simulink model "positionloop1"  (R2024a)
settings: Solver=FixedStepAuto  StartTime=0.0  StopTime=10  FixedStep=1e-4  RelTol=1e-3
values from neighbouring files (symbols this model uses):
  CurrKi = 35.0    [positionloop.sldd]
  CurrKp = 0.17    [positionloop.sldd]
  J = 9.6E-6    [positionloop.sldd]
  Ke = 0.076394372684109757    [positionloop.sldd]
  Kt = 0.132    [positionloop.sldd]
  L = 0.00179    [positionloop.sldd]
  Pn = 8.0    [positionloop.sldd]
  Rs = 1.93    [positionloop.sldd]
  SpdKi = 0.0144    [positionloop.sldd]
  SpdKp = 0.3389    [positionloop.sldd]
  Ts = 0.0001    [positionloop.sldd]
  Udc = 48.0    [positionloop.sldd]
undefined symbols (not defined in the file or in its folder): curr_q_ki, curr_q_kp, I, Jm, K, k_b, k_t, Kd
libraries: slpidlib x33, simulink x8, mcbplantlib x6, autolibpmsmexterior x6, RCTblocks x2
(part 1 of 4)
settings Model: DataDictionary=positionloop.sldd  Creator=Administrator  LastModifiedBy=WuHongrui
settings OptimizationCC: DefaultParameterBehavior=Inlined  UseDivisionForNetSlopeComputation=on  GainParamInheritBuiltInType=on  UseFloatMulNetSlope=on  InlineInvariantSignals=on  PassReuseOutputArgsAs=Individual arguments  ZeroExternalMemoryAtStartup=off  ZeroInternalMemoryAtStartup=off  NoFixptDivByZeroProtection=on  EfficientFloat2IntCast=on  LifeSpan=1  OptimizeBlockOrder=speed  DifferentSizesBufferReuse=on  EfficientTunableParamExpr=on
settings DebuggingCC: ParameterTunabilityLossMsg=error  UnconnectedInputMsg=warning  UnconnectedOutputMsg=warning  UnconnectedLineMsg=warning
settings HardwareCC: ProdBitPerPointer=32  ProdBitPerSizeT=32  ProdBitPerPtrDiffT=32  ProdLargestAtomicInteger=Long  ProdLargestAtomicFloat=Double  ProdWordSize=32  ProdLongLongMode=on  ProdHWDeviceType=ARM Compatible->ARM Cortex-M
settings ModelReferenceCC: EnableRefExpFcnMdlSchedulingChecks=on
settings SFSimCC: MATLABDynamicMemAlloc=off
settings RTWCC: Description=Embedded Coder  SystemTargetFile=ert.tlc  GenCodeOnly=on  PackageGeneratedCodeAndArtifacts=on  TemplateMakefile=ert_default_tmf  GenerateReport=on  LaunchReport=on  GenerateCodeReplacementReport=on  GPUComputeCapability=3.5  DLArmComputeVersion=19.05
settings CodeAppCC: ForceParamTrailComments=on  IgnoreCustomStorageClasses=off  OperatorAnnotations=on  SimulinkDataObjDesc=on  SFDataObjDesc=on  CustomSymbolStrGlobalVar=rt$N$M  CustomSymbolStrType=$N$M  CustomSymbolStrFcn=$N$M$F  CustomSymbolStrMacro=$N$M  InsertBlockDesc=on
settings ERTTargetCC: TargetLangStandard=C99 (ISO)  CodeReplacementLibrary=ARM Cortex-M  GenerateSampleERTMain=on  IncludeMdlTerminateFcn=off  CombineSignalStateStructs=on  SuppressErrorStatus=on  SupportComplex=off  InlinedParameterPlacement=NonHierarchical  ERTCustomFileTemplate=example_file_process.tlc  ERTFilePackagingFormat=CompactWithDataFile

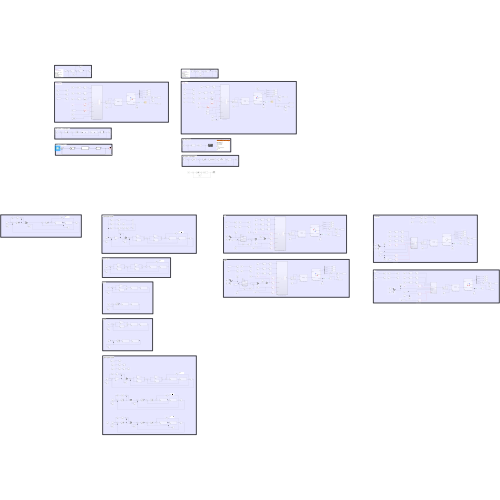
[thumbnail: Simulink's stored preview of the top-level diagram]
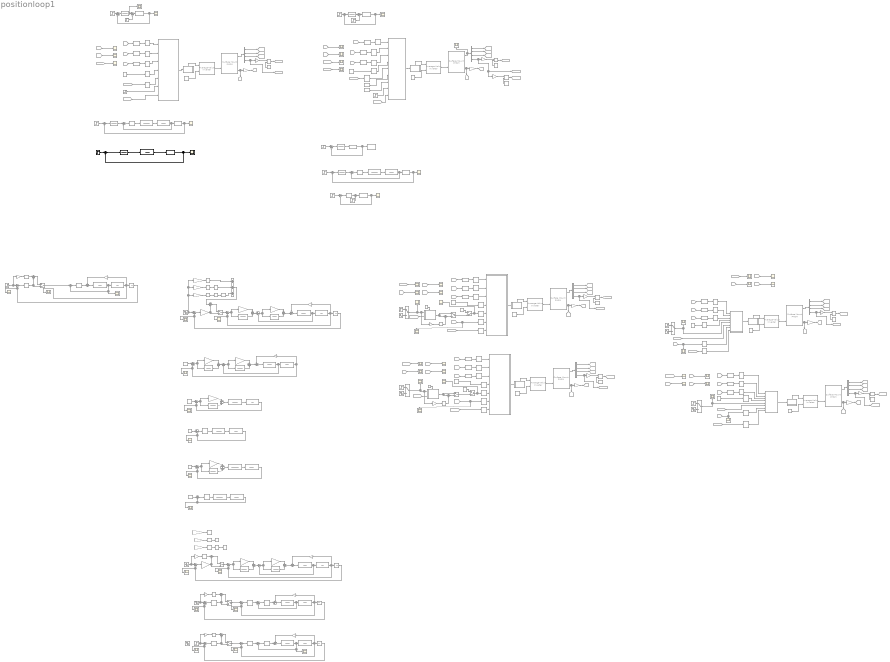
== system positionloop1 ==
  note: 三环
  note: 速度环
  note: S imulate Multiple Random Samples
      | vals = struct();
      | mdl = "positionloop";
      | open_system(mdl);
      | uvars = ufind(mdl);
      | n = 5;
      | for i=1:n
      | vals = usample(uvars);
      | sim(mdl);
      | end
  note: Ke = $\frac{3}{100\pi}Ke^{'}$
  note: Ke = $\frac{3}{100\pi}Ke^{'}$
  note: Ke = $\frac{3}{100\pi}Ke^{'}$
  note: Ke = $\frac{3}{100\pi}Ke^{'}$
  note: 电流环
  note: 速度环+电流环
  note: 位置环+速度环+电流环
  note: 整定
  note: 鲁棒+电流环（考虑减速器？）
  note: 未整定
  note: 系统不确定性仿真
  note: 鲁棒控制
      | （考虑减速器）
      |
      | 执行该仿真前，请打开MATLAB的 mu_synthesis.mlx 文件，运行到第56行，
      | [不确定性参数]之前。
  note: 鲁棒控制
      | （考虑减速器）
  note: 三环+前馈
  note: Ke = $\frac{3}{100\pi}Ke^{'}$
  note: 位置环+速度环+电流环
  note: Ke = $\frac{3}{100\pi}Ke^{'}$
  note: 鲁棒控制
      | （不考虑减速器）
      |
      | 执行该仿真前，请打开MATLAB的 mu_synthesis.mlx 文件，运行到第56行，
      | [不确定性参数]之前。
  note: 鲁棒控制
      | （不考虑减速器）
  note: 鲁棒+电流环（不考虑减速器）
  note: 鲁棒（不考虑减速器）
  Add : Sum  Commented=on  Inputs=+++
  Average-Value Inverter{1..6} (6 alike) : mcbplantlib/Average-Value Inverter  Commented=on
  Bus Selector{1..6} (6 alike) : BusSelector  Commented=on  OutputSignals=IaStator,IbStator,IcStator,MtrPos
  Constant1 : Constant  Commented=on  Value=1.5
  Constant{7,10,12,15,18,21} (6 alike) : Constant  Commented=on  Value=Udc
  Constant{8,11,13,16,19,22} (6 alike) : Constant  Commented=on  Value=Udc  OutDataTypeStr=single
  Constant{5,9,14,17,20,23..24} (7 alike) : Constant  Commented=on  Value=2*pi  OutDataTypeStr=single
  Constant2 : Constant  Commented=on  Value=300
  Constant25 : Constant  Commented=on  Value=0.1  OutDataTypeStr=single
  Constant26 : Constant  Commented=on  Value=0  OutDataTypeStr=single
  Constant3 : Constant  Commented=on
  Constant4 : Constant  Commented=on  Value=300
  Constant6 : Constant  Commented=on  Value=300
  Data Type Conversion{1..9,12..20} (18 alike) : DataTypeConversion  Commented=on  OutDataTypeStr=single  SaturateOnIntegerOverflow=off  RndMeth=Floor
  Derivative{1..18} (18 alike) : Derivative  Commented=on
  From{1,10,13,26,36,48} (6 alike) : From  Commented=on  GotoTag=theta_e  TagVisibility=global
  From{2,9,11,22,30..31,37,40,47,50,57} (11 alike) : From  Commented=on  GotoTag=theta_m  TagVisibility=global
  From{5,12,14,18,23,28,39,43,49,53} (10 alike) : From  Commented=on  GotoTag=W0
  From15 : From  Commented=on  GotoTag=theta_output  TagVisibility=global
  From{3,16,24,32,41,51} (6 alike) : From  Commented=on  GotoTag=ib
  From{4,17,25,33,42,52} (6 alike) : From  Commented=on  GotoTag=ic
  From{6,19,27,34,44,54} (6 alike) : From  Commented=on  GotoTag=Wm
  From{7,20,45,55} (4 alike) : From  Commented=on  GotoTag=theta
  From{8,21,29,35,46,56} (6 alike) : From  Commented=on  GotoTag=ia
  From58 : From  Commented=on  GotoTag=theta_output  TagVisibility=global
  Function-Call Generator1 : simulink/Ports & Subsystems/Function-Call Generator  Commented=on  sample_time=1e-2  numberOfIterations=1  DisallowWideOutput=off
  Function-Call Generator2 : simulink/Ports & Subsystems/Function-Call Generator  Commented=on  sample_time=1e-2  numberOfIterations=1  DisallowWideOutput=off
  Gain{,12..14,17,29} (6 alike) : Gain  Commented=on
  Gain{1,4,10,36} (4 alike) : Gain  Commented=on  Gain=CurrKp
  Gain11 : Gain  Commented=on  Gain=10
  Gain{6..7,15..16,37,39} (6 alike) : Gain  Commented=on  Gain=Ke
  Gain{2,18,20..21,25,27} (6 alike) : Gain  Commented=on  Gain=30/pi  OutDataTypeStr=single
  Gain{3,19,22..23,26,28} (6 alike) : Gain  Commented=on  Gain=Pn  OutDataTypeStr=single
  Gain24 : Gain  Commented=on  Gain=10
  Gain30 : Gain  Commented=on  Gain=L*J/Kt
  Gain31 : Gain  Commented=on  Gain=L*J/Kt
  Gain32 : Gain  Commented=on  Gain=Rs*J/Kt
  Gain33 : Gain  Commented=on  Gain=(Kt+Ke)/Kt
  Gain34 : Gain  Commented=on  Gain=Rs*J/Kt
  Gain35 : Gain  Commented=on  Gain=(Kt+Ke)/Kt
  Gain{5,8..9,38} (4 alike) : Gain  Commented=on  Gain=SpdKp
  Gain40 : Gain  Commented=on  Gain=80  OutDataTypeStr=single
  Goto{,3,12,18,32,39} (6 alike) : Goto  Commented=on  GotoTag=theta_m  TagVisibility=global
  Goto{1,10,15,22,29,36} (6 alike) : Goto  Commented=on  GotoTag=theta_e  TagVisibility=global
  Goto{2,11,17,24,31,38} (6 alike) : Goto  Commented=on  GotoTag=Wm
  Goto{4,13,19,26,33,40} (6 alike) : Goto  Commented=on  GotoTag=W0
  Goto{9,14,16,23,30,37} (6 alike) : Goto  Commented=on  GotoTag=ic
  Goto{5,7,20,27,34,41} (6 alike) : Goto  Commented=on  GotoTag=ia
  Goto{6,8,21,28,35,42} (6 alike) : Goto  Commented=on  GotoTag=ib
  Goto43 : Goto  Commented=on  GotoTag=theta_output  TagVisibility=global
  Integrator{,1..4} (5 alike) : Integrator  Commented=on
  Manual Switch{,1..2,5..8,11..13} (10 alike) : ManualSwitch  Commented=on
  Manual Switch14 : ManualSwitch  Commented=on  CurrentSetting=0
  Manual Switch3 : ManualSwitch  Commented=on  CurrentSetting=0
  Manual Switch4 : ManualSwitch  Commented=on  CurrentSetting=0
  Mod{1..7} (7 alike) : Math  Commented=on  Operator=mod  OutputSignalType=real
  MultiPlot Graph : RCTblocks/MultiPlot Graph  Tag=MultiPlot  Commented=on  tmin=0  tmax=5  ymin=0  ymax=2  vnamesave=multisimout
  PID Controller : slpidlib/PID Controller  Commented=on  Controller=PID  Form=Parallel  TimeDomain=Continuous-time  UseExternalTs=off  SampleTime=-1  IntegratorMethod=Forward Euler  FilterMethod=Forward Euler  ControllerParametersSource=internal  P=0.186  I=0  UseKiTs=off  D=0.087  UseExternalDerivativeSource=off  N=24686.714732734  UseFilter=on  TunerSelectOption=Transfer Function Based (PID Tuner App)  InitialConditionSource=internal  InitialConditionForIntegrator=0  InitialConditionForFilter=0  DifferentiatorICPrevScaledInput=0  ExternalReset=none  TrackingMode=off  Kt=1  LimitOutput=on  SatLimitsSource=internal  UpperSaturationLimit=10  LowerSaturationLimit=-10  LinearizeAsGain=on  AntiWindupMode=none  Kb=1  LimitIntegrator=off  UpperIntegratorSaturationLimit=inf  LowerIntegratorSaturationLimit=-inf  POutMin=[]  POutMax=[]  IOutMin=[]  IOutMax=[]  DOutMin=[]  DOutMax=[]  NOutMin=[]  NOutMax=[]  SumOutMin=[]  SumOutMax=[]  SaturationOutMin=[]  SaturationOutMax=[]  PParamMin=[]  PParamMax=[]  IParamMin=[]  IParamMax=[]  DParamMin=[]  DParamMax=[]  NParamMin=[]  NParamMax=[]  KbParamMin=[]  KbParamMax=[]  KtParamMin=[]  KtParamMax=[]  KbOutMin=[]  KbOutMax=[]  KtOutMin=[]  KtOutMax=[]  IntegratorOutMin=[]  IntegratorOutMax=[]  FilterOutMin=[]  FilterOutMax=[]  SumI1OutMin=[]  SumI1OutMax=[]  SumI2OutMin=[]  SumI2OutMax=[]  SumI3OutMin=[]  SumI3OutMax=[]  SumI4OutMin=[]  SumI4OutMax=[]  SumDOutMin=[]  SumDOutMax=[]  DifferentiatorOutMin=[]  DifferentiatorOutMax=[]  FilterDiffOutCoefMin=[]  FilterDiffOutCoefMax=[]  ReciprocalOutMin=[]  ReciprocalOutMax=[]  SumDenOutMin=[]  SumDenOutMax=[]  SumNumOutMin=[]  SumNumOutMax=[]  DivideOutMin=[]  DivideOutMax=[]  UdiffTsProdOutMin=[]  UdiffTsProdOutMax=[]  NTsProdOutMin=[]  NTsProdOutMax=[]  UintegralTsProdOutMin=[]  UintegralTsProdOutMax=[]  UngainTsProdOutMin=[]  UngainTsProdOutMax=[]  ClampingZeroOutDataTypeStr=Inherit: Inherit via back propagation  ClampingZeroOutMin=[]  ClampingZeroOutMax=[]  FilterDenConstantOutDataTypeStr=Inherit: Inherit via back propagation  FilterDenConstantOutMin=[]  FilterDenConstantOutMax=[]  PCopyOutDataTypeStr=Inherit: Inherit via back propagation  PCopyOutMin=[]  PCopyOutMax=[]  NCopyOutDataTypeStr=Inherit: Inherit via back propagation  NCopyOutMin=[]  NCopyOutMax=[]  IntegratorContinuousStateAttributes=''  IntegratorStateMustResolveToSignalObject=off  IntegratorRTWStateStorageClass=Auto  FilterContinuousStateAttributes=''  FilterStateMustResolveToSignalObject=off  FilterRTWStateStorageClass=Auto  ParallelPVariant=InternalParameters  IdealPVariant=Disabled  IVariant=InternalParameters  DVariant=InternalParameters  IntegratorVariant=Continuous  SatVariant=Enabled  AWVariant=Passthrough  PCopyVariant=Disabled  TRVariant=Disabled  FdbkBlocksVariant=Forward  IdealPFdbkVariant=Disabled  SatFdbkVariant=Disabled  DerivativeFilterVariant=ContFilter  NVariant=InternalParameters  NCopyVariant=Disabled  FilterICVariant=InternalICsFilter  IntegratorICVariant=InternalICs  ExternalResetVariant=Disabled  TRSumVariant=Passthrough  SumFdbkVariant=Disabled  SumVariant=Sum_PID  TsampFilterVariant=InternalTs  TsampNgainVariant=Passthrough  TsampIntegralVariant=Disabled_SignalSpec  ExternalSaturationOutDataTypeStr=Inherit: Same as second input  DerivativeSourceVariant=ErrorSignal
  PID Controller1 : slpidlib/PID Controller  Commented=on  Controller=PI  Form=Parallel  TimeDomain=Continuous-time  UseExternalTs=off  SampleTime=-1  IntegratorMethod=Forward Euler  FilterMethod=Forward Euler  ControllerParametersSource=internal  P=SpdKp  I=SpdKi  UseKiTs=off  D=0  UseExternalDerivativeSource=off  N=100  UseFilter=on  TunerSelectOption=Transfer Function Based (PID Tuner App)  InitialConditionSource=internal  InitialConditionForIntegrator=0  InitialConditionForFilter=0  DifferentiatorICPrevScaledInput=0  ExternalReset=none  TrackingMode=off  Kt=1  LimitOutput=on  SatLimitsSource=internal  UpperSaturationLimit=10  LowerSaturationLimit=-10  LinearizeAsGain=on  AntiWindupMode=none  Kb=1  LimitIntegrator=off  UpperIntegratorSaturationLimit=inf  LowerIntegratorSaturationLimit=-inf  POutMin=[]  POutMax=[]  IOutMin=[]  IOutMax=[]  DOutMin=[]  DOutMax=[]  NOutMin=[]  NOutMax=[]  SumOutMin=[]  SumOutMax=[]  SaturationOutMin=[]  SaturationOutMax=[]  PParamMin=[]  PParamMax=[]  IParamMin=[]  IParamMax=[]  DParamMin=[]  DParamMax=[]  NParamMin=[]  NParamMax=[]  KbParamMin=[]  KbParamMax=[]  KtParamMin=[]  KtParamMax=[]  KbOutMin=[]  KbOutMax=[]  KtOutMin=[]  KtOutMax=[]  IntegratorOutMin=[]  IntegratorOutMax=[]  FilterOutMin=[]  FilterOutMax=[]  SumI1OutMin=[]  SumI1OutMax=[]  SumI2OutMin=[]  SumI2OutMax=[]  SumI3OutMin=[]  SumI3OutMax=[]  SumI4OutMin=[]  SumI4OutMax=[]  SumDOutMin=[]  SumDOutMax=[]  DifferentiatorOutMin=[]  DifferentiatorOutMax=[]  FilterDiffOutCoefMin=[]  FilterDiffOutCoefMax=[]  ReciprocalOutMin=[]  ReciprocalOutMax=[]  SumDenOutMin=[]  SumDenOutMax=[]  SumNumOutMin=[]  SumNumOutMax=[]  DivideOutMin=[]  DivideOutMax=[]  UdiffTsProdOutMin=[]  UdiffTsProdOutMax=[]  NTsProdOutMin=[]  NTsProdOutMax=[]  UintegralTsProdOutMin=[]  UintegralTsProdOutMax=[]  UngainTsProdOutMin=[]  UngainTsProdOutMax=[]  ClampingZeroOutDataTypeStr=Inherit: Inherit via back propagation  ClampingZeroOutMin=[]  ClampingZeroOutMax=[]  FilterDenConstantOutDataTypeStr=Inherit: Inherit via back propagation  FilterDenConstantOutMin=[]  FilterDenConstantOutMax=[]  PCopyOutDataTypeStr=Inherit: Inherit via back propagation  PCopyOutMin=[]  PCopyOutMax=[]  NCopyOutDataTypeStr=Inherit: Inherit via back propagation  NCopyOutMin=[]  NCopyOutMax=[]  IntegratorContinuousStateAttributes=''  IntegratorStateMustResolveToSignalObject=off  IntegratorRTWStateStorageClass=Auto  FilterContinuousStateAttributes=''  FilterStateMustResolveToSignalObject=off  FilterRTWStateStorageClass=Auto  ParallelPVariant=InternalParameters  IdealPVariant=Disabled  IVariant=InternalParameters  DVariant=Disabled  IntegratorVariant=Continuous  SatVariant=Enabled  AWVariant=Passthrough  PCopyVariant=Disabled  TRVariant=Disabled  FdbkBlocksVariant=Forward  IdealPFdbkVariant=Disabled  SatFdbkVariant=Disabled  DerivativeFilterVariant=Disabled  NVariant=Disabled  NCopyVariant=Disabled_SignalSpec  FilterICVariant=Disabled  IntegratorICVariant=InternalICs  ExternalResetVariant=Disabled  TRSumVariant=Passthrough  SumFdbkVariant=Disabled  SumVariant=Sum_PI  TsampFilterVariant=InternalTs  TsampNgainVariant=Passthrough  TsampIntegralVariant=Disabled_SignalSpec  ExternalSaturationOutDataTypeStr=Inherit: Same as second input  DerivativeSourceVariant=Disabled
  PID Controller10 : slpidlib/PID Controller  Commented=on  Controller=P  Form=Parallel  TimeDomain=Continuous-time  UseExternalTs=off  SampleTime=-1  IntegratorMethod=Forward Euler  FilterMethod=Forward Euler  ControllerParametersSource=internal  P=14.0449429845648  I=1.40448915956441e-06  UseKiTs=off  D=0  UseExternalDerivativeSource=off  N=100  UseFilter=on  TunerSelectOption=Transfer Function Based (PID Tuner App)  InitialConditionSource=internal  InitialConditionForIntegrator=0  InitialConditionForFilter=0  DifferentiatorICPrevScaledInput=0  ExternalReset=none  TrackingMode=off  Kt=1  LimitOutput=on  SatLimitsSource=internal  UpperSaturationLimit=Udc*0.9/sqrt(3)  LowerSaturationLimit=-Udc*0.9/sqrt(3)  LinearizeAsGain=on  AntiWindupMode=none  Kb=1  LimitIntegrator=off  UpperIntegratorSaturationLimit=inf  LowerIntegratorSaturationLimit=-inf  POutMin=[]  POutMax=[]  IOutMin=[]  IOutMax=[]  DOutMin=[]  DOutMax=[]  NOutMin=[]  NOutMax=[]  SumOutMin=[]  SumOutMax=[]  SaturationOutMin=[]  SaturationOutMax=[]  PParamMin=[]  PParamMax=[]  IParamMin=[]  IParamMax=[]  DParamMin=[]  DParamMax=[]  NParamMin=[]  NParamMax=[]  KbParamMin=[]  KbParamMax=[]  KtParamMin=[]  KtParamMax=[]  KbOutMin=[]  KbOutMax=[]  KtOutMin=[]  KtOutMax=[]  IntegratorOutMin=[]  IntegratorOutMax=[]  FilterOutMin=[]  FilterOutMax=[]  SumI1OutMin=[]  SumI1OutMax=[]  SumI2OutMin=[]  SumI2OutMax=[]  SumI3OutMin=[]  SumI3OutMax=[]  SumI4OutMin=[]  SumI4OutMax=[]  SumDOutMin=[]  SumDOutMax=[]  DifferentiatorOutMin=[]  DifferentiatorOutMax=[]  FilterDiffOutCoefMin=[]  FilterDiffOutCoefMax=[]  ReciprocalOutMin=[]  ReciprocalOutMax=[]  SumDenOutMin=[]  SumDenOutMax=[]  SumNumOutMin=[]  SumNumOutMax=[]  DivideOutMin=[]  DivideOutMax=[]  UdiffTsProdOutMin=[]  UdiffTsProdOutMax=[]  NTsProdOutMin=[]  NTsProdOutMax=[]  UintegralTsProdOutMin=[]  UintegralTsProdOutMax=[]  UngainTsProdOutMin=[]  UngainTsProdOutMax=[]  ClampingZeroOutDataTypeStr=Inherit: Inherit via back propagation  ClampingZeroOutMin=[]  ClampingZeroOutMax=[]  FilterDenConstantOutDataTypeStr=Inherit: Inherit via back propagation  FilterDenConstantOutMin=[]  FilterDenConstantOutMax=[]  PCopyOutDataTypeStr=Inherit: Inherit via back propagation  PCopyOutMin=[]  PCopyOutMax=[]  NCopyOutDataTypeStr=Inherit: Inherit via back propagation  NCopyOutMin=[]  NCopyOutMax=[]  IntegratorContinuousStateAttributes=''  IntegratorStateMustResolveToSignalObject=off  IntegratorRTWStateStorageClass=Auto  FilterContinuousStateAttributes=''  FilterStateMustResolveToSignalObject=off  FilterRTWStateStorageClass=Auto  ParallelPVariant=InternalParameters  IdealPVariant=Disabled  IVariant=Disabled  DVariant=Disabled  IntegratorVariant=Disabled  SatVariant=Enabled  AWVariant=Disabled  PCopyVariant=Disabled  TRVariant=Disabled  FdbkBlocksVariant=Forward  IdealPFdbkVariant=Disabled  SatFdbkVariant=Disabled  DerivativeFilterVariant=Disabled  NVariant=Disabled  NCopyVariant=Disabled_SignalSpec  FilterICVariant=Disabled  IntegratorICVariant=Disabled  ExternalResetVariant=Disabled  TRSumVariant=Passthrough  SumFdbkVariant=Disabled  SumVariant=Passthrough_P  TsampFilterVariant=InternalTs  TsampNgainVariant=Passthrough  TsampIntegralVariant=Disabled_SignalSpec  ExternalSaturationOutDataTypeStr=Inherit: Same as second input  DerivativeSourceVariant=Disabled
  PID Controller12 : slpidlib/PID Controller  Commented=on  Controller=PI  Form=Parallel  TimeDomain=Continuous-time  UseExternalTs=off  SampleTime=-1  IntegratorMethod=Forward Euler  FilterMethod=Forward Euler  ControllerParametersSource=internal  P=0.0444061130539005  I=8.20535972466433e-05  UseKiTs=off  D=0  UseExternalDerivativeSource=off  N=100  UseFilter=on  TunerSelectOption=Transfer Function Based (PID Tuner App)  InitialConditionSource=internal  InitialConditionForIntegrator=0  InitialConditionForFilter=0  DifferentiatorICPrevScaledInput=0  ExternalReset=none  TrackingMode=off  Kt=1  LimitOutput=on  SatLimitsSource=internal  UpperSaturationLimit=Udc*0.9/sqrt(3)  LowerSaturationLimit=-Udc*0.9/sqrt(3)  LinearizeAsGain=on  AntiWindupMode=none  Kb=1  LimitIntegrator=off  UpperIntegratorSaturationLimit=inf  LowerIntegratorSaturationLimit=-inf  POutMin=[]  POutMax=[]  IOutMin=[]  IOutMax=[]  DOutMin=[]  DOutMax=[]  NOutMin=[]  NOutMax=[]  SumOutMin=[]  SumOutMax=[]  SaturationOutMin=[]  SaturationOutMax=[]  PParamMin=[]  PParamMax=[]  IParamMin=[]  IParamMax=[]  DParamMin=[]  DParamMax=[]  NParamMin=[]  NParamMax=[]  KbParamMin=[]  KbParamMax=[]  KtParamMin=[]  KtParamMax=[]  KbOutMin=[]  KbOutMax=[]  KtOutMin=[]  KtOutMax=[]  IntegratorOutMin=[]  IntegratorOutMax=[]  FilterOutMin=[]  FilterOutMax=[]  SumI1OutMin=[]  SumI1OutMax=[]  SumI2OutMin=[]  SumI2OutMax=[]  SumI3OutMin=[]  SumI3OutMax=[]  SumI4OutMin=[]  SumI4OutMax=[]  SumDOutMin=[]  SumDOutMax=[]  DifferentiatorOutMin=[]  DifferentiatorOutMax=[]  FilterDiffOutCoefMin=[]  FilterDiffOutCoefMax=[]  ReciprocalOutMin=[]  ReciprocalOutMax=[]  SumDenOutMin=[]  SumDenOutMax=[]  SumNumOutMin=[]  SumNumOutMax=[]  DivideOutMin=[]  DivideOutMax=[]  UdiffTsProdOutMin=[]  UdiffTsProdOutMax=[]  NTsProdOutMin=[]  NTsProdOutMax=[]  UintegralTsProdOutMin=[]  UintegralTsProdOutMax=[]  UngainTsProdOutMin=[]  UngainTsProdOutMax=[]  ClampingZeroOutDataTypeStr=Inherit: Inherit via back propagation  ClampingZeroOutMin=[]  ClampingZeroOutMax=[]  FilterDenConstantOutDataTypeStr=Inherit: Inherit via back propagation  FilterDenConstantOutMin=[]  FilterDenConstantOutMax=[]  PCopyOutDataTypeStr=Inherit: Inherit via back propagation  PCopyOutMin=[]  PCopyOutMax=[]  NCopyOutDataTypeStr=Inherit: Inherit via back propagation  NCopyOutMin=[]  NCopyOutMax=[]  IntegratorContinuousStateAttributes=''  IntegratorStateMustResolveToSignalObject=off  IntegratorRTWStateStorageClass=Auto  FilterContinuousStateAttributes=''  FilterStateMustResolveToSignalObject=off  FilterRTWStateStorageClass=Auto  ParallelPVariant=InternalParameters  IdealPVariant=Disabled  IVariant=InternalParameters  DVariant=Disabled  IntegratorVariant=Continuous  SatVariant=Enabled  AWVariant=Passthrough  PCopyVariant=Disabled  TRVariant=Disabled  FdbkBlocksVariant=Forward  IdealPFdbkVariant=Disabled  SatFdbkVariant=Disabled  DerivativeFilterVariant=Disabled  NVariant=Disabled  NCopyVariant=Disabled_SignalSpec  FilterICVariant=Disabled  IntegratorICVariant=InternalICs  ExternalResetVariant=Disabled  TRSumVariant=Passthrough  SumFdbkVariant=Disabled  SumVariant=Sum_PI  TsampFilterVariant=InternalTs  TsampNgainVariant=Passthrough  TsampIntegralVariant=Disabled_SignalSpec  ExternalSaturationOutDataTypeStr=Inherit: Same as second input  DerivativeSourceVariant=Disabled
  PID Controller13 : slpidlib/PID Controller  Commented=on  Controller=PI  Form=Parallel  TimeDomain=Continuous-time  UseExternalTs=off  SampleTime=-1  IntegratorMethod=Forward Euler  FilterMethod=Forward Euler  ControllerParametersSource=internal  P=3.78093167506926  I=4.06645918177242e-07  UseKiTs=off  D=0  UseExternalDerivativeSource=off  N=100  UseFilter=on  TunerSelectOption=Transfer Function Based (PID Tuner App)  InitialConditionSource=internal  InitialConditionForIntegrator=0  InitialConditionForFilter=0  DifferentiatorICPrevScaledInput=0  ExternalReset=none  TrackingMode=off  Kt=1  LimitOutput=on  SatLimitsSource=internal  UpperSaturationLimit=10  LowerSaturationLimit=-10  LinearizeAsGain=on  AntiWindupMode=none  Kb=1  LimitIntegrator=off  UpperIntegratorSaturationLimit=inf  LowerIntegratorSaturationLimit=-inf  POutMin=[]  POutMax=[]  IOutMin=[]  IOutMax=[]  DOutMin=[]  DOutMax=[]  NOutMin=[]  NOutMax=[]  SumOutMin=[]  SumOutMax=[]  SaturationOutMin=[]  SaturationOutMax=[]  PParamMin=[]  PParamMax=[]  IParamMin=[]  IParamMax=[]  DParamMin=[]  DParamMax=[]  NParamMin=[]  NParamMax=[]  KbParamMin=[]  KbParamMax=[]  KtParamMin=[]  KtParamMax=[]  KbOutMin=[]  KbOutMax=[]  KtOutMin=[]  KtOutMax=[]  IntegratorOutMin=[]  IntegratorOutMax=[]  FilterOutMin=[]  FilterOutMax=[]  SumI1OutMin=[]  SumI1OutMax=[]  SumI2OutMin=[]  SumI2OutMax=[]  SumI3OutMin=[]  SumI3OutMax=[]  SumI4OutMin=[]  SumI4OutMax=[]  SumDOutMin=[]  SumDOutMax=[]  DifferentiatorOutMin=[]  DifferentiatorOutMax=[]  FilterDiffOutCoefMin=[]  FilterDiffOutCoefMax=[]  ReciprocalOutMin=[]  ReciprocalOutMax=[]  SumDenOutMin=[]  SumDenOutMax=[]  SumNumOutMin=[]  SumNumOutMax=[]  DivideOutMin=[]  DivideOutMax=[]  UdiffTsProdOutMin=[]  UdiffTsProdOutMax=[]  NTsProdOutMin=[]  NTsProdOutMax=[]  UintegralTsProdOutMin=[]  UintegralTsProdOutMax=[]  UngainTsProdOutMin=[]  UngainTsProdOutMax=[]  ClampingZeroOutDataTypeStr=Inherit: Inherit via back propagation  ClampingZeroOutMin=[]  ClampingZeroOutMax=[]  FilterDenConstantOutDataTypeStr=Inherit: Inherit via back propagation  FilterDenConstantOutMin=[]  FilterDenConstantOutMax=[]  PCopyOutDataTypeStr=Inherit: Inherit via back propagation  PCopyOutMin=[]  PCopyOutMax=[]  NCopyOutDataTypeStr=Inherit: Inherit via back propagation  NCopyOutMin=[]  NCopyOutMax=[]  IntegratorContinuousStateAttributes=''  IntegratorStateMustResolveToSignalObject=off  IntegratorRTWStateStorageClass=Auto  FilterContinuousStateAttributes=''  FilterStateMustResolveToSignalObject=off  FilterRTWStateStorageClass=Auto  ParallelPVariant=InternalParameters  IdealPVariant=Disabled  IVariant=InternalParameters  DVariant=Disabled  IntegratorVariant=Continuous  SatVariant=Enabled  AWVariant=Passthrough  PCopyVariant=Disabled  TRVariant=Disabled  FdbkBlocksVariant=Forward  IdealPFdbkVariant=Disabled  SatFdbkVariant=Disabled  DerivativeFilterVariant=Disabled  NVariant=Disabled  NCopyVariant=Disabled_SignalSpec  FilterICVariant=Disabled  IntegratorICVariant=InternalICs  ExternalResetVariant=Disabled  TRSumVariant=Passthrough  SumFdbkVariant=Disabled  SumVariant=Sum_PI  TsampFilterVariant=InternalTs  TsampNgainVariant=Passthrough  TsampIntegralVariant=Disabled_SignalSpec  ExternalSaturationOutDataTypeStr=Inherit: Same as second input  DerivativeSourceVariant=Disabled
  PID Controller2 : slpidlib/PID Controller  Commented=on  Controller=PI  Form=Parallel  TimeDomain=Continuous-time  UseExternalTs=off  SampleTime=-1  IntegratorMethod=Forward Euler  FilterMethod=Forward Euler  ControllerParametersSource=internal  P=CurrKp  I=CurrKi  UseKiTs=off  D=0  UseExternalDerivativeSource=off  N=100  UseFilter=on  TunerSelectOption=Transfer Function Based (PID Tuner App)  InitialConditionSource=internal  InitialConditionForIntegrator=0  InitialConditionForFilter=0  DifferentiatorICPrevScaledInput=0  ExternalReset=none  TrackingMode=off  Kt=1  LimitOutput=on  SatLimitsSource=internal  UpperSaturationLimit=Udc*0.9/sqrt(3)  LowerSaturationLimit=-Udc*0.9/sqrt(3)  LinearizeAsGain=on  AntiWindupMode=none  Kb=1  LimitIntegrator=off  UpperIntegratorSaturationLimit=inf  LowerIntegratorSaturationLimit=-inf  POutMin=[]  POutMax=[]  IOutMin=[]  IOutMax=[]  DOutMin=[]  DOutMax=[]  NOutMin=[]  NOutMax=[]  SumOutMin=[]  SumOutMax=[]  SaturationOutMin=[]  SaturationOutMax=[]  PParamMin=[]  PParamMax=[]  IParamMin=[]  IParamMax=[]  DParamMin=[]  DParamMax=[]  NParamMin=[]  NParamMax=[]  KbParamMin=[]  KbParamMax=[]  KtParamMin=[]  KtParamMax=[]  KbOutMin=[]  KbOutMax=[]  KtOutMin=[]  KtOutMax=[]  IntegratorOutMin=[]  IntegratorOutMax=[]  FilterOutMin=[]  FilterOutMax=[]  SumI1OutMin=[]  SumI1OutMax=[]  SumI2OutMin=[]  SumI2OutMax=[]  SumI3OutMin=[]  SumI3OutMax=[]  SumI4OutMin=[]  SumI4OutMax=[]  SumDOutMin=[]  SumDOutMax=[]  DifferentiatorOutMin=[]  DifferentiatorOutMax=[]  FilterDiffOutCoefMin=[]  FilterDiffOutCoefMax=[]  ReciprocalOutMin=[]  ReciprocalOutMax=[]  SumDenOutMin=[]  SumDenOutMax=[]  SumNumOutMin=[]  SumNumOutMax=[]  DivideOutMin=[]  DivideOutMax=[]  UdiffTsProdOutMin=[]  UdiffTsProdOutMax=[]  NTsProdOutMin=[]  NTsProdOutMax=[]  UintegralTsProdOutMin=[]  UintegralTsProdOutMax=[]  UngainTsProdOutMin=[]  UngainTsProdOutMax=[]  ClampingZeroOutDataTypeStr=Inherit: Inherit via back propagation  ClampingZeroOutMin=[]  ClampingZeroOutMax=[]  FilterDenConstantOutDataTypeStr=Inherit: Inherit via back propagation  FilterDenConstantOutMin=[]  FilterDenConstantOutMax=[]  PCopyOutDataTypeStr=Inherit: Inherit via back propagation  PCopyOutMin=[]  PCopyOutMax=[]  NCopyOutDataTypeStr=Inherit: Inherit via back propagation  NCopyOutMin=[]  NCopyOutMax=[]  IntegratorContinuousStateAttributes=''  IntegratorStateMustResolveToSignalObject=off  IntegratorRTWStateStorageClass=Auto  FilterContinuousStateAttributes=''  FilterStateMustResolveToSignalObject=off  FilterRTWStateStorageClass=Auto  ParallelPVariant=InternalParameters  IdealPVariant=Disabled  IVariant=InternalParameters  DVariant=Disabled  IntegratorVariant=Continuous  SatVariant=Enabled  AWVariant=Passthrough  PCopyVariant=Disabled  TRVariant=Disabled  FdbkBlocksVariant=Forward  IdealPFdbkVariant=Disabled  SatFdbkVariant=Disabled  DerivativeFilterVariant=Disabled  NVariant=Disabled  NCopyVariant=Disabled_SignalSpec  FilterICVariant=Disabled  IntegratorICVariant=InternalICs  ExternalResetVariant=Disabled  TRSumVariant=Passthrough  SumFdbkVariant=Disabled  SumVariant=Sum_PI  TsampFilterVariant=InternalTs  TsampNgainVariant=Passthrough  TsampIntegralVariant=Disabled_SignalSpec  ExternalSaturationOutDataTypeStr=Inherit: Same as second input  DerivativeSourceVariant=Disabled
  PID Controller3 : slpidlib/PID Controller  Commented=on  Controller=P  Form=Parallel  TimeDomain=Continuous-time  UseExternalTs=off  SampleTime=-1  IntegratorMethod=Forward Euler  FilterMethod=Forward Euler  ControllerParametersSource=internal  P=10  I=SpdKi  UseKiTs=off  D=0  UseExternalDerivativeSource=off  N=100  UseFilter=on  TunerSelectOption=Transfer Function Based (PID Tuner App)  InitialConditionSource=internal  InitialConditionForIntegrator=0  InitialConditionForFilter=0  DifferentiatorICPrevScaledInput=0  ExternalReset=none  TrackingMode=off  Kt=1  LimitOutput=on  SatLimitsSource=internal  UpperSaturationLimit=400  LowerSaturationLimit=-400  LinearizeAsGain=on  AntiWindupMode=none  Kb=1  LimitIntegrator=off  UpperIntegratorSaturationLimit=inf  LowerIntegratorSaturationLimit=-inf  POutMin=[]  POutMax=[]  IOutMin=[]  IOutMax=[]  DOutMin=[]  DOutMax=[]  NOutMin=[]  NOutMax=[]  SumOutMin=[]  SumOutMax=[]  SaturationOutMin=[]  SaturationOutMax=[]  PParamMin=[]  PParamMax=[]  IParamMin=[]  IParamMax=[]  DParamMin=[]  DParamMax=[]  NParamMin=[]  NParamMax=[]  KbParamMin=[]  KbParamMax=[]  KtParamMin=[]  KtParamMax=[]  KbOutMin=[]  KbOutMax=[]  KtOutMin=[]  KtOutMax=[]  IntegratorOutMin=[]  IntegratorOutMax=[]  FilterOutMin=[]  FilterOutMax=[]  SumI1OutMin=[]  SumI1OutMax=[]  SumI2OutMin=[]  SumI2OutMax=[]  SumI3OutMin=[]  SumI3OutMax=[]  SumI4OutMin=[]  SumI4OutMax=[]  SumDOutMin=[]  SumDOutMax=[]  DifferentiatorOutMin=[]  DifferentiatorOutMax=[]  FilterDiffOutCoefMin=[]  FilterDiffOutCoefMax=[]  ReciprocalOutMin=[]  ReciprocalOutMax=[]  SumDenOutMin=[]  SumDenOutMax=[]  SumNumOutMin=[]  SumNumOutMax=[]  DivideOutMin=[]  DivideOutMax=[]  UdiffTsProdOutMin=[]  UdiffTsProdOutMax=[]  NTsProdOutMin=[]  NTsProdOutMax=[]  UintegralTsProdOutMin=[]  UintegralTsProdOutMax=[]  UngainTsProdOutMin=[]  UngainTsProdOutMax=[]  ClampingZeroOutDataTypeStr=Inherit: Inherit via back propagation  ClampingZeroOutMin=[]  ClampingZeroOutMax=[]  FilterDenConstantOutDataTypeStr=Inherit: Inherit via back propagation  FilterDenConstantOutMin=[]  FilterDenConstantOutMax=[]  PCopyOutDataTypeStr=Inherit: Inherit via back propagation  PCopyOutMin=[]  PCopyOutMax=[]  NCopyOutDataTypeStr=Inherit: Inherit via back propagation  NCopyOutMin=[]  NCopyOutMax=[]  IntegratorContinuousStateAttributes=''  IntegratorStateMustResolveToSignalObject=off  IntegratorRTWStateStorageClass=Auto  FilterContinuousStateAttributes=''  FilterStateMustResolveToSignalObject=off  FilterRTWStateStorageClass=Auto  ParallelPVariant=InternalParameters  IdealPVariant=Disabled  IVariant=Disabled  DVariant=Disabled  IntegratorVariant=Disabled  SatVariant=Enabled  AWVariant=Disabled  PCopyVariant=Disabled  TRVariant=Disabled  FdbkBlocksVariant=Forward  IdealPFdbkVariant=Disabled  SatFdbkVariant=Disabled  DerivativeFilterVariant=Disabled  NVariant=Disabled  NCopyVariant=Disabled_SignalSpec  FilterICVariant=Disabled  IntegratorICVariant=Disabled  ExternalResetVariant=Disabled  TRSumVariant=Passthrough  SumFdbkVariant=Disabled  SumVariant=Passthrough_P  TsampFilterVariant=InternalTs  TsampNgainVariant=Passthrough  TsampIntegralVariant=Disabled_SignalSpec  ExternalSaturationOutDataTypeStr=Inherit: Same as second input  DerivativeSourceVariant=Disabled
  PID Controller4 : slpidlib/PID Controller  Commented=on  Controller=PI  Form=Parallel  TimeDomain=Continuous-time  UseExternalTs=off  SampleTime=-1  IntegratorMethod=Forward Euler  FilterMethod=Forward Euler  ControllerParametersSource=internal  P=0.515264878487547  I=987.649638453674  UseKiTs=off  D=0  UseExternalDerivativeSource=off  N=100  UseFilter=on  TunerSelectOption=Transfer Function Based (PID Tuner App)  InitialConditionSource=internal  InitialConditionForIntegrator=0  InitialConditionForFilter=0  DifferentiatorICPrevScaledInput=0  ExternalReset=none  TrackingMode=off  Kt=1  LimitOutput=on  SatLimitsSource=internal  UpperSaturationLimit=Udc*0.9/sqrt(3)  LowerSaturationLimit=-Udc*0.9/sqrt(3)  LinearizeAsGain=on  AntiWindupMode=none  Kb=1  LimitIntegrator=off  UpperIntegratorSaturationLimit=inf  LowerIntegratorSaturationLimit=-inf  POutMin=[]  POutMax=[]  IOutMin=[]  IOutMax=[]  DOutMin=[]  DOutMax=[]  NOutMin=[]  NOutMax=[]  SumOutMin=[]  SumOutMax=[]  SaturationOutMin=[]  SaturationOutMax=[]  PParamMin=[]  PParamMax=[]  IParamMin=[]  IParamMax=[]  DParamMin=[]  DParamMax=[]  NParamMin=[]  NParamMax=[]  KbParamMin=[]  KbParamMax=[]  KtParamMin=[]  KtParamMax=[]  KbOutMin=[]  KbOutMax=[]  KtOutMin=[]  KtOutMax=[]  IntegratorOutMin=[]  IntegratorOutMax=[]  FilterOutMin=[]  FilterOutMax=[]  SumI1OutMin=[]  SumI1OutMax=[]  SumI2OutMin=[]  SumI2OutMax=[]  SumI3OutMin=[]  SumI3OutMax=[]  SumI4OutMin=[]  SumI4OutMax=[]  SumDOutMin=[]  SumDOutMax=[]  DifferentiatorOutMin=[]  DifferentiatorOutMax=[]  FilterDiffOutCoefMin=[]  FilterDiffOutCoefMax=[]  ReciprocalOutMin=[]  ReciprocalOutMax=[]  SumDenOutMin=[]  SumDenOutMax=[]  SumNumOutMin=[]  SumNumOutMax=[]  DivideOutMin=[]  DivideOutMax=[]  UdiffTsProdOutMin=[]  UdiffTsProdOutMax=[]  NTsProdOutMin=[]  NTsProdOutMax=[]  UintegralTsProdOutMin=[]  UintegralTsProdOutMax=[]  UngainTsProdOutMin=[]  UngainTsProdOutMax=[]  ClampingZeroOutDataTypeStr=Inherit: Inherit via back propagation  ClampingZeroOutMin=[]  ClampingZeroOutMax=[]  FilterDenConstantOutDataTypeStr=Inherit: Inherit via back propagation  FilterDenConstantOutMin=[]  FilterDenConstantOutMax=[]  PCopyOutDataTypeStr=Inherit: Inherit via back propagation  PCopyOutMin=[]  PCopyOutMax=[]  NCopyOutDataTypeStr=Inherit: Inherit via back propagation  NCopyOutMin=[]  NCopyOutMax=[]  IntegratorContinuousStateAttributes=''  IntegratorStateMustResolveToSignalObject=off  IntegratorRTWStateStorageClass=Auto  FilterContinuousStateAttributes=''  FilterStateMustResolveToSignalObject=off  FilterRTWStateStorageClass=Auto  ParallelPVariant=InternalParameters  IdealPVariant=Disabled  IVariant=InternalParameters  DVariant=Disabled  IntegratorVariant=Continuous  SatVariant=Enabled  AWVariant=Passthrough  PCopyVariant=Disabled  TRVariant=Disabled  FdbkBlocksVariant=Forward  IdealPFdbkVariant=Disabled  SatFdbkVariant=Disabled  DerivativeFilterVariant=Disabled  NVariant=Disabled  NCopyVariant=Disabled_SignalSpec  FilterICVariant=Disabled  IntegratorICVariant=InternalICs  ExternalResetVariant=Disabled  TRSumVariant=Passthrough  SumFdbkVariant=Disabled  SumVariant=Sum_PI  TsampFilterVariant=InternalTs  TsampNgainVariant=Passthrough  TsampIntegralVariant=Disabled_SignalSpec  ExternalSaturationOutDataTypeStr=Inherit: Same as second input  DerivativeSourceVariant=Disabled
  PID Controller5 : slpidlib/PID Controller  Commented=on  Controller=PI  Form=Parallel  TimeDomain=Continuous-time  UseExternalTs=off  SampleTime=-1  IntegratorMethod=Forward Euler  FilterMethod=Forward Euler  ControllerParametersSource=internal  P=0.0357379215593134  I=0.00228786760899636  UseKiTs=off  D=0  UseExternalDerivativeSource=off  N=100  UseFilter=on  TunerSelectOption=Transfer Function Based (PID Tuner App)  InitialConditionSource=internal  InitialConditionForIntegrator=0  InitialConditionForFilter=0  DifferentiatorICPrevScaledInput=0  ExternalReset=none  TrackingMode=off  Kt=1  LimitOutput=on  SatLimitsSource=internal  UpperSaturationLimit=10  LowerSaturationLimit=-10  LinearizeAsGain=on  AntiWindupMode=none  Kb=1  LimitIntegrator=off  UpperIntegratorSaturationLimit=inf  LowerIntegratorSaturationLimit=-inf  POutMin=[]  POutMax=[]  IOutMin=[]  IOutMax=[]  DOutMin=[]  DOutMax=[]  NOutMin=[]  NOutMax=[]  SumOutMin=[]  SumOutMax=[]  SaturationOutMin=[]  SaturationOutMax=[]  PParamMin=[]  PParamMax=[]  IParamMin=[]  IParamMax=[]  DParamMin=[]  DParamMax=[]  NParamMin=[]  NParamMax=[]  KbParamMin=[]  KbParamMax=[]  KtParamMin=[]  KtParamMax=[]  KbOutMin=[]  KbOutMax=[]  KtOutMin=[]  KtOutMax=[]  IntegratorOutMin=[]  IntegratorOutMax=[]  FilterOutMin=[]  FilterOutMax=[]  SumI1OutMin=[]  SumI1OutMax=[]  SumI2OutMin=[]  SumI2OutMax=[]  SumI3OutMin=[]  SumI3OutMax=[]  SumI4OutMin=[]  SumI4OutMax=[]  SumDOutMin=[]  SumDOutMax=[]  DifferentiatorOutMin=[]  DifferentiatorOutMax=[]  FilterDiffOutCoefMin=[]  FilterDiffOutCoefMax=[]  ReciprocalOutMin=[]  ReciprocalOutMax=[]  SumDenOutMin=[]  SumDenOutMax=[]  SumNumOutMin=[]  SumNumOutMax=[]  DivideOutMin=[]  DivideOutMax=[]  UdiffTsProdOutMin=[]  UdiffTsProdOutMax=[]  NTsProdOutMin=[]  NTsProdOutMax=[]  UintegralTsProdOutMin=[]  UintegralTsProdOutMax=[]  UngainTsProdOutMin=[]  UngainTsProdOutMax=[]  ClampingZeroOutDataTypeStr=Inherit: Inherit via back propagation  ClampingZeroOutMin=[]  ClampingZeroOutMax=[]  FilterDenConstantOutDataTypeStr=Inherit: Inherit via back propagation  FilterDenConstantOutMin=[]  FilterDenConstantOutMax=[]  PCopyOutDataTypeStr=Inherit: Inherit via back propagation  PCopyOutMin=[]  PCopyOutMax=[]  NCopyOutDataTypeStr=Inherit: Inherit via back propagation  NCopyOutMin=[]  NCopyOutMax=[]  IntegratorContinuousStateAttributes=''  IntegratorStateMustResolveToSignalObject=off  IntegratorRTWStateStorageClass=Auto  FilterContinuousStateAttributes=''  FilterStateMustResolveToSignalObject=off  FilterRTWStateStorageClass=Auto  ParallelPVariant=InternalParameters  IdealPVariant=Disabled  IVariant=InternalParameters  DVariant=Disabled  IntegratorVariant=Continuous  SatVariant=Enabled  AWVariant=Passthrough  PCopyVariant=Disabled  TRVariant=Disabled  FdbkBlocksVariant=Forward  IdealPFdbkVariant=Disabled  SatFdbkVariant=Disabled  DerivativeFilterVariant=Disabled  NVariant=Disabled  NCopyVariant=Disabled_SignalSpec  FilterICVariant=Disabled  IntegratorICVariant=InternalICs  ExternalResetVariant=Disabled  TRSumVariant=Passthrough  SumFdbkVariant=Disabled  SumVariant=Sum_PI  TsampFilterVariant=InternalTs  TsampNgainVariant=Passthrough  TsampIntegralVariant=Disabled_SignalSpec  ExternalSaturationOutDataTypeStr=Inherit: Same as second input  DerivativeSourceVariant=Disabled
  PID Controller6 : slpidlib/PID Controller  Commented=on  Controller=PI  Form=Parallel  TimeDomain=Continuous-time  UseExternalTs=off  SampleTime=-1  IntegratorMethod=Forward Euler  FilterMethod=Forward Euler  ControllerParametersSource=internal  P=0.0357379215593134  I=0.00228786760899636  UseKiTs=off  D=0  UseExternalDerivativeSource=off  N=100  UseFilter=on  TunerSelectOption=Transfer Function Based (PID Tuner App)  InitialConditionSource=internal  InitialConditionForIntegrator=0  InitialConditionForFilter=0  DifferentiatorICPrevScaledInput=0  ExternalReset=none  TrackingMode=off  Kt=1  LimitOutput=on  SatLimitsSource=internal  UpperSaturationLimit=10  LowerSaturationLimit=-10  LinearizeAsGain=on  AntiWindupMode=none  Kb=1  LimitIntegrator=off  UpperIntegratorSaturationLimit=inf  LowerIntegratorSaturationLimit=-inf  POutMin=[]  POutMax=[]  IOutMin=[]  IOutMax=[]  DOutMin=[]  DOutMax=[]  NOutMin=[]  NOutMax=[]  SumOutMin=[]  SumOutMax=[]  SaturationOutMin=[]  SaturationOutMax=[]  PParamMin=[]  PParamMax=[]  IParamMin=[]  IParamMax=[]  DParamMin=[]  DParamMax=[]  NParamMin=[]  NParamMax=[]  KbParamMin=[]  KbParamMax=[]  KtParamMin=[]  KtParamMax=[]  KbOutMin=[]  KbOutMax=[]  KtOutMin=[]  KtOutMax=[]  IntegratorOutMin=[]  IntegratorOutMax=[]  FilterOutMin=[]  FilterOutMax=[]  SumI1OutMin=[]  SumI1OutMax=[]  SumI2OutMin=[]  SumI2OutMax=[]  SumI3OutMin=[]  SumI3OutMax=[]  SumI4OutMin=[]  SumI4OutMax=[]  SumDOutMin=[]  SumDOutMax=[]  DifferentiatorOutMin=[]  DifferentiatorOutMax=[]  FilterDiffOutCoefMin=[]  FilterDiffOutCoefMax=[]  ReciprocalOutMin=[]  ReciprocalOutMax=[]  SumDenOutMin=[]  SumDenOutMax=[]  SumNumOutMin=[]  SumNumOutMax=[]  DivideOutMin=[]  DivideOutMax=[]  UdiffTsProdOutMin=[]  UdiffTsProdOutMax=[]  NTsProdOutMin=[]  NTsProdOutMax=[]  UintegralTsProdOutMin=[]  UintegralTsProdOutMax=[]  UngainTsProdOutMin=[]  UngainTsProdOutMax=[]  ClampingZeroOutDataTypeStr=Inherit: Inherit via back propagation  ClampingZeroOutMin=[]  ClampingZeroOutMax=[]  FilterDenConstantOutDataTypeStr=Inherit: Inherit via back propagation  FilterDenConstantOutMin=[]  FilterDenConstantOutMax=[]  PCopyOutDataTypeStr=Inherit: Inherit via back propagation  PCopyOutMin=[]  PCopyOutMax=[]  NCopyOutDataTypeStr=Inherit: Inherit via back propagation  NCopyOutMin=[]  NCopyOutMax=[]  IntegratorContinuousStateAttributes=''  IntegratorStateMustResolveToSignalObject=off  IntegratorRTWStateStorageClass=Auto  FilterContinuousStateAttributes=''  FilterStateMustResolveToSignalObject=off  FilterRTWStateStorageClass=Auto  ParallelPVariant=InternalParameters  IdealPVariant=Disabled  IVariant=InternalParameters  DVariant=Disabled  IntegratorVariant=Continuous  SatVariant=Enabled  AWVariant=Passthrough  PCopyVariant=Disabled  TRVariant=Disabled  FdbkBlocksVariant=Forward  IdealPFdbkVariant=Disabled  SatFdbkVariant=Disabled  DerivativeFilterVariant=Disabled  NVariant=Disabled  NCopyVariant=Disabled_SignalSpec  FilterICVariant=Disabled  IntegratorICVariant=InternalICs  ExternalResetVariant=Disabled  TRSumVariant=Passthrough  SumFdbkVariant=Disabled  SumVariant=Sum_PI  TsampFilterVariant=InternalTs  TsampNgainVariant=Passthrough  TsampIntegralVariant=Disabled_SignalSpec  ExternalSaturationOutDataTypeStr=Inherit: Same as second input  DerivativeSourceVariant=Disabled
  PID Controller7 : slpidlib/PID Controller  Commented=on  Controller=PI  Form=Parallel  TimeDomain=Continuous-time  UseExternalTs=off  SampleTime=-1  IntegratorMethod=Forward Euler  FilterMethod=Forward Euler  ControllerParametersSource=internal  P=140761.099230136  I=0.0289367750531912  UseKiTs=off  D=0  UseExternalDerivativeSource=off  N=100  UseFilter=on  TunerSelectOption=Transfer Function Based (PID Tuner App)  InitialConditionSource=internal  InitialConditionForIntegrator=0  InitialConditionForFilter=0  DifferentiatorICPrevScaledInput=0  ExternalReset=none  TrackingMode=off  Kt=1  LimitOutput=on  SatLimitsSource=internal  UpperSaturationLimit=Udc*0.9/sqrt(3)  LowerSaturationLimit=-Udc*0.9/sqrt(3)  LinearizeAsGain=on  AntiWindupMode=none  Kb=1  LimitIntegrator=off  UpperIntegratorSaturationLimit=inf  LowerIntegratorSaturationLimit=-inf  POutMin=[]  POutMax=[]  IOutMin=[]  IOutMax=[]  DOutMin=[]  DOutMax=[]  NOutMin=[]  NOutMax=[]  SumOutMin=[]  SumOutMax=[]  SaturationOutMin=[]  SaturationOutMax=[]  PParamMin=[]  PParamMax=[]  IParamMin=[]  IParamMax=[]  DParamMin=[]  DParamMax=[]  NParamMin=[]  NParamMax=[]  KbParamMin=[]  KbParamMax=[]  KtParamMin=[]  KtParamMax=[]  KbOutMin=[]  KbOutMax=[]  KtOutMin=[]  KtOutMax=[]  IntegratorOutMin=[]  IntegratorOutMax=[]  FilterOutMin=[]  FilterOutMax=[]  SumI1OutMin=[]  SumI1OutMax=[]  SumI2OutMin=[]  SumI2OutMax=[]  SumI3OutMin=[]  SumI3OutMax=[]  SumI4OutMin=[]  SumI4OutMax=[]  SumDOutMin=[]  SumDOutMax=[]  DifferentiatorOutMin=[]  DifferentiatorOutMax=[]  FilterDiffOutCoefMin=[]  FilterDiffOutCoefMax=[]  ReciprocalOutMin=[]  ReciprocalOutMax=[]  SumDenOutMin=[]  SumDenOutMax=[]  SumNumOutMin=[]  SumNumOutMax=[]  DivideOutMin=[]  DivideOutMax=[]  UdiffTsProdOutMin=[]  UdiffTsProdOutMax=[]  NTsProdOutMin=[]  NTsProdOutMax=[]  UintegralTsProdOutMin=[]  UintegralTsProdOutMax=[]  UngainTsProdOutMin=[]  UngainTsProdOutMax=[]  ClampingZeroOutDataTypeStr=Inherit: Inherit via back propagation  ClampingZeroOutMin=[]  ClampingZeroOutMax=[]  FilterDenConstantOutDataTypeStr=Inherit: Inherit via back propagation  FilterDenConstantOutMin=[]  FilterDenConstantOutMax=[]  PCopyOutDataTypeStr=Inherit: Inherit via back propagation  PCopyOutMin=[]  PCopyOutMax=[]  NCopyOutDataTypeStr=Inherit: Inherit via back propagation  NCopyOutMin=[]  NCopyOutMax=[]  IntegratorContinuousStateAttributes=''  IntegratorStateMustResolveToSignalObject=off  IntegratorRTWStateStorageClass=Auto  FilterContinuousStateAttributes=''  FilterStateMustResolveToSignalObject=off  FilterRTWStateStorageClass=Auto  ParallelPVariant=InternalParameters  IdealPVariant=Disabled  IVariant=InternalParameters  DVariant=Disabled  IntegratorVariant=Continuous  SatVariant=Enabled  AWVariant=Passthrough  PCopyVariant=Disabled  TRVariant=Disabled  FdbkBlocksVariant=Forward  IdealPFdbkVariant=Disabled  SatFdbkVariant=Disabled  DerivativeFilterVariant=Disabled  NVariant=Disabled  NCopyVariant=Disabled_SignalSpec  FilterICVariant=Disabled  IntegratorICVariant=InternalICs  ExternalResetVariant=Disabled  TRSumVariant=Passthrough  SumFdbkVariant=Disabled  SumVariant=Sum_PI  TsampFilterVariant=InternalTs  TsampNgainVariant=Passthrough  TsampIntegralVariant=Disabled_SignalSpec  ExternalSaturationOutDataTypeStr=Inherit: Same as second input  DerivativeSourceVariant=Disabled
  PID Controller8 : slpidlib/PID Controller  Commented=on  Controller=P  Form=Parallel  TimeDomain=Continuous-time  UseExternalTs=off  SampleTime=-1  IntegratorMethod=Forward Euler  FilterMethod=Forward Euler  ControllerParametersSource=internal  P=49.3058532817775  I=SpdKi  UseKiTs=off  D=0  UseExternalDerivativeSource=off  N=100  UseFilter=on  TunerSelectOption=Transfer Function Based (PID Tuner App)  InitialConditionSource=internal  InitialConditionForIntegrator=0  InitialConditionForFilter=0  DifferentiatorICPrevScaledInput=0  ExternalReset=none  TrackingMode=off  Kt=1  LimitOutput=on  SatLimitsSource=internal  UpperSaturationLimit=400  LowerSaturationLimit=-400  LinearizeAsGain=on  AntiWindupMode=none  Kb=1  LimitIntegrator=off  UpperIntegratorSaturationLimit=inf  LowerIntegratorSaturationLimit=-inf  POutMin=[]  POutMax=[]  IOutMin=[]  IOutMax=[]  DOutMin=[]  DOutMax=[]  NOutMin=[]  NOutMax=[]  SumOutMin=[]  SumOutMax=[]  SaturationOutMin=[]  SaturationOutMax=[]  PParamMin=[]  PParamMax=[]  IParamMin=[]  IParamMax=[]  DParamMin=[]  DParamMax=[]  NParamMin=[]  NParamMax=[]  KbParamMin=[]  KbParamMax=[]  KtParamMin=[]  KtParamMax=[]  KbOutMin=[]  KbOutMax=[]  KtOutMin=[]  KtOutMax=[]  IntegratorOutMin=[]  IntegratorOutMax=[]  FilterOutMin=[]  FilterOutMax=[]  SumI1OutMin=[]  SumI1OutMax=[]  SumI2OutMin=[]  SumI2OutMax=[]  SumI3OutMin=[]  SumI3OutMax=[]  SumI4OutMin=[]  SumI4OutMax=[]  SumDOutMin=[]  SumDOutMax=[]  DifferentiatorOutMin=[]  DifferentiatorOutMax=[]  FilterDiffOutCoefMin=[]  FilterDiffOutCoefMax=[]  ReciprocalOutMin=[]  ReciprocalOutMax=[]  SumDenOutMin=[]  SumDenOutMax=[]  SumNumOutMin=[]  SumNumOutMax=[]  DivideOutMin=[]  DivideOutMax=[]  UdiffTsProdOutMin=[]  UdiffTsProdOutMax=[]  NTsProdOutMin=[]  NTsProdOutMax=[]  UintegralTsProdOutMin=[]  UintegralTsProdOutMax=[]  UngainTsProdOutMin=[]  UngainTsProdOutMax=[]  ClampingZeroOutDataTypeStr=Inherit: Inherit via back propagation  ClampingZeroOutMin=[]  ClampingZeroOutMax=[]  FilterDenConstantOutDataTypeStr=Inherit: Inherit via back propagation  FilterDenConstantOutMin=[]  FilterDenConstantOutMax=[]  PCopyOutDataTypeStr=Inherit: Inherit via back propagation  PCopyOutMin=[]  PCopyOutMax=[]  NCopyOutDataTypeStr=Inherit: Inherit via back propagation  NCopyOutMin=[]  NCopyOutMax=[]  IntegratorContinuousStateAttributes=''  IntegratorStateMustResolveToSignalObject=off  IntegratorRTWStateStorageClass=Auto  FilterContinuousStateAttributes=''  FilterStateMustResolveToSignalObject=off  FilterRTWStateStorageClass=Auto  ParallelPVariant=InternalParameters  IdealPVariant=Disabled  IVariant=Disabled  DVariant=Disabled  IntegratorVariant=Disabled  SatVariant=Enabled  AWVariant=Disabled  PCopyVariant=Disabled  TRVariant=Disabled  FdbkBlocksVariant=Forward  IdealPFdbkVariant=Disabled  SatFdbkVariant=Disabled  DerivativeFilterVariant=Disabled  NVariant=Disabled  NCopyVariant=Disabled_SignalSpec  FilterICVariant=Disabled  IntegratorICVariant=Disabled  ExternalResetVariant=Disabled  TRSumVariant=Passthrough  SumFdbkVariant=Disabled  SumVariant=Passthrough_P  TsampFilterVariant=InternalTs  TsampNgainVariant=Passthrough  TsampIntegralVariant=Disabled_SignalSpec  ExternalSaturationOutDataTypeStr=Inherit: Same as second input  DerivativeSourceVariant=Disabled
  PID Controller9 : slpidlib/PID Controller  Commented=on  Controller=PI  Form=Parallel  TimeDomain=Continuous-time  UseExternalTs=off  SampleTime=-1  IntegratorMethod=Forward Euler  FilterMethod=Forward Euler  ControllerParametersSource=internal  P=0.515264878487547  I=987.649638453674  UseKiTs=off  D=0  UseExternalDerivativeSource=off  N=100  UseFilter=on  TunerSelectOption=Transfer Function Based (PID Tuner App)  InitialConditionSource=internal  InitialConditionForIntegrator=0  InitialConditionForFilter=0  DifferentiatorICPrevScaledInput=0  ExternalReset=none  TrackingMode=off  Kt=1  LimitOutput=on  SatLimitsSource=internal  UpperSaturationLimit=Udc*0.9/sqrt(3)  LowerSaturationLimit=-Udc*0.9/sqrt(3)  LinearizeAsGain=on  AntiWindupMode=none  Kb=1  LimitIntegrator=off  UpperIntegratorSaturationLimit=inf  LowerIntegratorSaturationLimit=-inf  POutMin=[]  POutMax=[]  IOutMin=[]  IOutMax=[]  DOutMin=[]  DOutMax=[]  NOutMin=[]  NOutMax=[]  SumOutMin=[]  SumOutMax=[]  SaturationOutMin=[]  SaturationOutMax=[]  PParamMin=[]  PParamMax=[]  IParamMin=[]  IParamMax=[]  DParamMin=[]  DParamMax=[]  NParamMin=[]  NParamMax=[]  KbParamMin=[]  KbParamMax=[]  KtParamMin=[]  KtParamMax=[]  KbOutMin=[]  KbOutMax=[]  KtOutMin=[]  KtOutMax=[]  IntegratorOutMin=[]  IntegratorOutMax=[]  FilterOutMin=[]  FilterOutMax=[]  SumI1OutMin=[]  SumI1OutMax=[]  SumI2OutMin=[]  SumI2OutMax=[]  SumI3OutMin=[]  SumI3OutMax=[]  SumI4OutMin=[]  SumI4OutMax=[]  SumDOutMin=[]  SumDOutMax=[]  DifferentiatorOutMin=[]  DifferentiatorOutMax=[]  FilterDiffOutCoefMin=[]  FilterDiffOutCoefMax=[]  ReciprocalOutMin=[]  ReciprocalOutMax=[]  SumDenOutMin=[]  SumDenOutMax=[]  SumNumOutMin=[]  SumNumOutMax=[]  DivideOutMin=[]  DivideOutMax=[]  UdiffTsProdOutMin=[]  UdiffTsProdOutMax=[]  NTsProdOutMin=[]  NTsProdOutMax=[]  UintegralTsProdOutMin=[]  UintegralTsProdOutMax=[]  UngainTsProdOutMin=[]  UngainTsProdOutMax=[]  ClampingZeroOutDataTypeStr=Inherit: Inherit via back propagation  ClampingZeroOutMin=[]  ClampingZeroOutMax=[]  FilterDenConstantOutDataTypeStr=Inherit: Inherit via back propagation  FilterDenConstantOutMin=[]  FilterDenConstantOutMax=[]  PCopyOutDataTypeStr=Inherit: Inherit via back propagation  PCopyOutMin=[]  PCopyOutMax=[]  NCopyOutDataTypeStr=Inherit: Inherit via back propagation  NCopyOutMin=[]  NCopyOutMax=[]  IntegratorContinuousStateAttributes=''  IntegratorStateMustResolveToSignalObject=off  IntegratorRTWStateStorageClass=Auto  FilterContinuousStateAttributes=''  FilterStateMustResolveToSignalObject=off  FilterRTWStateStorageClass=Auto  ParallelPVariant=InternalParameters  IdealPVariant=Disabled  IVariant=InternalParameters  DVariant=Disabled  IntegratorVariant=Continuous  SatVariant=Enabled  AWVariant=Passthrough  PCopyVariant=Disabled  TRVariant=Disabled  FdbkBlocksVariant=Forward  IdealPFdbkVariant=Disabled  SatFdbkVariant=Disabled  DerivativeFilterVariant=Disabled  NVariant=Disabled  NCopyVariant=Disabled_SignalSpec  FilterICVariant=Disabled  IntegratorICVariant=InternalICs  ExternalResetVariant=Disabled  TRSumVariant=Passthrough  SumFdbkVariant=Disabled  SumVariant=Sum_PI  TsampFilterVariant=InternalTs  TsampNgainVariant=Passthrough  TsampIntegralVariant=Disabled_SignalSpec  ExternalSaturationOutDataTypeStr=Inherit: Same as second input  DerivativeSourceVariant=Disabled
  PositionLoop1 : Subsystem  Commented=on
  PositionLoop2 : Subsystem  Commented=on
  Rate Transition{1..11,13..21,23..33,35..39} (36 alike) : RateTransition  Commented=on
  Robust control : Subsystem  Commented=on  TreatAsAtomicUnit=on
  Scope{,1..56} (57 alike) : Scope  Commented=on
  Scope57 : Scope
  Sine Wave{1,3..4,10} (4 alike) : Sin  Commented=on  Amplitude=pi/2  Frequency=5  SampleTime=0
  Sine Wave{2,5,8..9} (4 alike) : Sin  Commented=on  Amplitude=pi/2  Frequency=5  SampleTime=1e-2
  Speed and Current Loop1 : Subsystem  Commented=on  TreatAsAtomicUnit=on
  Speed and Current Loop2 : Subsystem  Commented=on  TreatAsAtomicUnit=on
  Speed and Current Loop4 : Subsystem  Commented=on  TreatAsAtomicUnit=on
  State-Space{,2..4} (4 alike) : StateSpace  Commented=on  A=[0 1; 0 (-k_b*I-Kd)/(Jm*I)]  B=[0; k_t/(Jm*I)]  C=[1 0]  D=0  InitialCondition=0
  State-Space1 : StateSpace  Commented=on  A=[0 1; 0 (-k_b*I-K)/(Jm*I)]  B=[0; k_t/(Jm*I)]  C=[1 0]  D=0  InitialCondition=0
  State-Space5 : StateSpace  A=[0 1; 0 (-k_b*I-Kd)/(Jm*I)]  B=[0; k_t/(Jm*I)]  C=[1 0]  D=0  InitialCondition=0
  Step{1,3..5,12..13,17} (7 alike) : Step  Commented=on  Time=0  After=pi/3  SampleTime=1e-2
  Step10 : Step  Commented=on  Time=0  SampleTime=1e-2
  Step11 : Step  Commented=on  Time=0  SampleTime=1e-2
  Step{2,6,9,14..15} (5 alike) : Step  Commented=on  Time=0  After=2*pi  SampleTime=1e-2
  Step16 : Step  Commented=on  Time=0  After=pi  SampleTime=1e-2
  Step18 : Step  Time=0  After=pi/3  SampleTime=1e-3
  Step7 : Step  Commented=on  Time=0  After=pi  SampleTime=1e-2
  Step8 : Step  Commented=on  Time=0  After=0  SampleTime=1e-2
  Subsystem1 : Subsystem  Commented=on
      settings: PortSchema="{\"entries\":[{\"content\":{\"sides\":[{\"content\":{\"connectorIds\":[\"In1\"]},\"type\":\"ConnectorPlacement.EquallySpacedRectSide\",\"uuid\":\"8ccc51de-fa2a-4900-80a3-4cdf9aa76f01\"},{\"content\":{\"connectorIds\":[],\"side\":\"RIGHT\"},\"type\":\"ConnectorPlacement.EquallySpacedRectSide\",\"uuid\":\"32c06e0d-3f1d-4948-af96-e310e54308a0\"},{\"content\":{\"connectorIds\":[\"Out1\"],\"side\":\"TOP\"},\"type\":\"ConnectorPlacement.EquallySpacedRectSide\",\"uuid\":\"a9066067-2c54-42a8-b4d7-fb86ac71b860\"}]},\"type\":\"ConnectorPlacement.EquallySpacedConnector\",\"uuid\":\"e4576975-acad-4e16-822f-2c2e7f23d7a7\"}],\"packageUris\":[\"http://schema.mathworks.com/mf0/Connector/R2020b\"],\"version\":\"1.0\"}"
  Subsystem2 : Subsystem  Commented=on
      settings: PortSchema="{\"entries\":[{\"content\":{\"sides\":[{\"content\":{\"connectorIds\":[\"In1\"]},\"type\":\"ConnectorPlacement.EquallySpacedRectSide\",\"uuid\":\"8ccc51de-fa2a-4900-80a3-4cdf9aa76f01\"},{\"content\":{\"connectorIds\":[],\"side\":\"RIGHT\"},\"type\":\"ConnectorPlacement.EquallySpacedRectSide\",\"uuid\":\"32c06e0d-3f1d-4948-af96-e310e54308a0\"},{\"content\":{\"connectorIds\":[\"Out1\"],\"side\":\"TOP\"},\"type\":\"ConnectorPlacement.EquallySpacedRectSide\",\"uuid\":\"a9066067-2c54-42a8-b4d7-fb86ac71b860\"}]},\"type\":\"ConnectorPlacement.EquallySpacedConnector\",\"uuid\":\"e4576975-acad-4e16-822f-2c2e7f23d7a7\"}],\"packageUris\":[\"http://schema.mathworks.com/mf0/Connector/R2020b\"],\"version\":\"1.0\"}"
  Subsystem3 : Subsystem  Commented=on
      settings: PortSchema="{\"entries\":[{\"content\":{\"sides\":[{\"content\":{\"connectorIds\":[\"In1\"]},\"type\":\"ConnectorPlacement.EquallySpacedRectSide\",\"uuid\":\"8ccc51de-fa2a-4900-80a3-4cdf9aa76f01\"},{\"content\":{\"connectorIds\":[],\"side\":\"RIGHT\"},\"type\":\"ConnectorPlacement.EquallySpacedRectSide\",\"uuid\":\"32c06e0d-3f1d-4948-af96-e310e54308a0\"},{\"content\":{\"connectorIds\":[\"Out1\"],\"side\":\"TOP\"},\"type\":\"ConnectorPlacement.EquallySpacedRectSide\",\"uuid\":\"a9066067-2c54-42a8-b4d7-fb86ac71b860\"}]},\"type\":\"ConnectorPlacement.EquallySpacedConnector\",\"uuid\":\"e4576975-acad-4e16-822f-2c2e7f23d7a7\"}],\"packageUris\":[\"http://schema.mathworks.com/mf0/Connector/R2020b\"],\"version\":\"1.0\"}"
  Subsystem4 : Subsystem  Commented=on
      settings: PortSchema="{\"entries\":[{\"content\":{\"sides\":[{\"content\":{\"connectorIds\":[\"In1\"]},\"type\":\"ConnectorPlacement.EquallySpacedRectSide\",\"uuid\":\"8ccc51de-fa2a-4900-80a3-4cdf9aa76f01\"},{\"content\":{\"connectorIds\":[],\"side\":\"RIGHT\"},\"type\":\"ConnectorPlacement.EquallySpacedRectSide\",\"uuid\":\"32c06e0d-3f1d-4948-af96-e310e54308a0\"},{\"content\":{\"connectorIds\":[\"Out1\"],\"side\":\"TOP\"},\"type\":\"ConnectorPlacement.EquallySpacedRectSide\",\"uuid\":\"a9066067-2c54-42a8-b4d7-fb86ac71b860\"}]},\"type\":\"ConnectorPlacement.EquallySpacedConnector\",\"uuid\":\"e4576975-acad-4e16-822f-2c2e7f23d7a7\"}],\"packageUris\":[\"http://schema.mathworks.com/mf0/Connector/R2020b\"],\"version\":\"1.0\"}"
  Subsystem5 : Subsystem  Commented=on
      settings: PortSchema="{\"entries\":[{\"content\":{\"sides\":[{\"content\":{\"connectorIds\":[\"In1\"]},\"type\":\"ConnectorPlacement.EquallySpacedRectSide\",\"uuid\":\"8ccc51de-fa2a-4900-80a3-4cdf9aa76f01\"},{\"content\":{\"connectorIds\":[],\"side\":\"RIGHT\"},\"type\":\"ConnectorPlacement.EquallySpacedRectSide\",\"uuid\":\"32c06e0d-3f1d-4948-af96-e310e54308a0\"},{\"content\":{\"connectorIds\":[\"Out1\"],\"side\":\"TOP\"},\"type\":\"ConnectorPlacement.EquallySpacedRectSide\",\"uuid\":\"a9066067-2c54-42a8-b4d7-fb86ac71b860\"}]},\"type\":\"ConnectorPlacement.EquallySpacedConnector\",\"uuid\":\"e4576975-acad-4e16-822f-2c2e7f23d7a7\"}],\"packageUris\":[\"http://schema.mathworks.com/mf0/Connector/R2020b\"],\"version\":\"1.0\"}"
  Subsystem6 : Subsystem  Commented=on
  Subsystem7 : Subsystem  Commented=on
      settings: PortSchema="{\"entries\":[{\"content\":{\"sides\":[{\"content\":{\"connectorIds\":[\"In1\"]},\"type\":\"ConnectorPlacement.EquallySpacedRectSide\",\"uuid\":\"8ccc51de-fa2a-4900-80a3-4cdf9aa76f01\"},{\"content\":{\"connectorIds\":[],\"side\":\"RIGHT\"},\"type\":\"ConnectorPlacement.EquallySpacedRectSide\",\"uuid\":\"32c06e0d-3f1d-4948-af96-e310e54308a0\"},{\"content\":{\"connectorIds\":[\"Out1\"],\"side\":\"TOP\"},\"type\":\"ConnectorPlacement.EquallySpacedRectSide\",\"uuid\":\"a9066067-2c54-42a8-b4d7-fb86ac71b860\"}]},\"type\":\"ConnectorPlacement.EquallySpacedConnector\",\"uuid\":\"e4576975-acad-4e16-822f-2c2e7f23d7a7\"}],\"packageUris\":[\"http://schema.mathworks.com/mf0/Connector/R2020b\"],\"version\":\"1.0\"}"
  Sum{,3,5,7,9,11,15..16,18..22,25..26,29,31..37,40..41,44..46,49..51} (31 alike) : Sum  Commented=on  Inputs=|+-
  Sum{1,17,23,27,30,42,47} (7 alike) : Sum  Commented=on  Inputs=|++
  Sum{6,10,24,28,43,48} (6 alike) : Sum  Commented=on  Inputs=-+|
  Sum{2,4,8,12..14,38..39} (8 alike) : Sum  Commented=on
  Sum52 : Sum  Inputs=|+-
  Surface Mount PMSM{1..6} (6 alike) : autolibpmsmexterior/Surface Mount PMSM  Commented=on  port_config=Torque  sim_type=Discrete  Ts=1e-4  P=Pn  Rs=Rs  Ldq_=L  KConstText=Torque constant (Kt):  lambda_pm=flux  Ke=0.0059268  Kt=Kt  mechanical=[0.096e-4, 2e-5, 0]  idq0=[0 0]  theta_init=0  omega_init=0  KConst=Kt  lambda_pm_calc=0.011  RefBlkName='autolibpmsmexterior/Surface Mount PMSM'  aMode=5  Ldq="[0.0017      0.0017]"
  Transfer Fcn{1,3,23,29} (4 alike) : TransferFcn  Commented=on  Denominator=[1.5*Ts 1]
  Transfer Fcn{8,10,14,17,20..21,31,35} (8 alike) : TransferFcn  Commented=on  Numerator=[Kt]  Denominator=[J 0]
  Transfer Fcn{9,11,15,32} (4 alike) : TransferFcn  Commented=on  Numerator=[SpdKi]  Denominator=[1 0]
  Transfer Fcn{2,4,12,16,19,22,24,30,33,36} (10 alike) : TransferFcn  Commented=on  Denominator=[L Rs]
  Transfer Fcn{5..6,13,34} (4 alike) : TransferFcn  Commented=on  Numerator=[CurrKi]  Denominator=[1 0]
  Transfer Fcn18 : TransferFcn  Commented=on  Denominator=[3*Ts 1]
  Transfer Fcn25 : TransferFcn  Commented=on  Numerator=[208.2 444.9]  Denominator=[1 74.06 2150]
  Transfer Fcn26 : TransferFcn  Commented=on  Numerator=[2.492e04, 8.681e05, 8.229e05]  Denominator=[1, 1.394e04, 3.159e06, 3.181e04]
  Transfer Fcn27 : TransferFcn  Commented=on  Numerator=[208.2 444.9]  Denominator=[1 74.06 2150]
  Transfer Fcn28 : TransferFcn  Commented=on  Numerator=[1.321e04, 4631]  Denominator=[1, 1.006e04, 101.9]
  Transfer Fcn37 : TransferFcn  Commented=on  Numerator=[2.492e04, 8.681e05, 8.229e05]  Denominator=[1, 1.394e04, 3.159e06, 3.181e04]
  Transfer Fcn39 : TransferFcn  Denominator=[L Rs]
  Transfer Fcn40 : TransferFcn  Numerator=[1.831e04, 1.064e05, 3.156e05]  Denominator=[1, 1.415e04, 2.716e06, 2.764e04]
  Transfer Fcn7 : TransferFcn  Commented=on  Denominator=[3*Ts 1]
  Triloop_Feedforward : Subsystem  Commented=on  TreatAsAtomicUnit=on
      settings: RTWSystemCode=Nonreusable function
  Uncertain State Space : RCTblocks/Uncertain State Space  Tag=USS  Commented=on  USystem=uss1  UValue=vals  X0=[]  uX0=[]
  rad/s1 : Constant  Commented=on  Value=183
  rad/s2 : Constant  Commented=on  Value=183
  wires:
  Sine Wave2/1 -> Manual Switch5/2
  Function-Call Generator2/1 -> PositionLoop2/Trigger
  Surface Mount PMSM1/1 -> Bus Selector1/1
  Step3/1 -> Manual Switch5/1
  From17/1 -> Data Type Conversion5/1
  Constant5/1 -> Mod3/2
  rad/s1/1 -> Manual Switch4/1
  From11/1 -> PositionLoop2/2(PositionFd)
  Rate Transition8/1 -> Speed and Current Loop1/1(ia)
  Constant7/1 -> Average-Value Inverter1/2
  Rate Transition16/1 -> Speed and Current Loop1/6(SpeedFd)
  From16/1 -> Data Type Conversion4/1
  Mod3/1 -> Goto10/1
  Bus Selector1/3 -> Goto9/1  "<IcStator>"
  From21/1 -> Data Type Conversion3/1
  From10/1 -> Rate Transition21/1
  Subsystem1/1(DutyOut) -> Average-Value Inverter1/1
  Bus Selector1/2 -> Goto8/1  "<IbStator>"
  Rate Transition15/1 -> Speed and Current Loop1/4(v_bus)
  Rate Transition13/1 -> Speed and Current Loop1/5(SpeedRef)
  Speed and Current Loop1/1(tABC) -> Subsystem1/1(DutyIn)
  Data Type Conversion4/1 -> Rate Transition9/1
  Rate Transition9/1 -> Speed and Current Loop1/2(ib)
  Gain3/1 -> Mod3/1
  Data Type Conversion5/1 -> Rate Transition10/1
  Average-Value Inverter1/1 -> Surface Mount PMSM1/2
  Rate Transition10/1 -> Speed and Current Loop1/3(ic)
  Bus Selector1/1 -> Goto7/1  "<IaStator>"
  Rate Transition21/1 -> Speed and Current Loop1/7(theta)
  Constant8/1 -> Rate Transition15/1
  Data Type Conversion3/1 -> Rate Transition8/1
  Gain2/1 -> Goto11/1
  From20/1 -> Scope11/1
  From19/1 -> Scope19/1
  Manual Switch6/1 -> Manual Switch4/2
  Sum1/1 -> Manual Switch6/2
  From22/1 -> Scope21/1
  From23/1 -> Scope13/1
  Derivative1/1 -> Sum1/2
  Gain/1 -> Derivative1/1
  Gain1/1 -> Sum2/1
  Transfer Fcn5/1 -> Sum2/2
  Sum2/1 -> Transfer Fcn3/1
  Sum3/1 -> Gain1/1, Transfer Fcn5/1
  Transfer Fcn4/1 -> Sum3/2, Scope/1
  Constant1/1 -> Sum3/1
  Transfer Fcn3/1 -> Transfer Fcn4/1
  Sum4/1 -> Transfer Fcn7/1
  Gain5/1 -> Sum4/1
  Constant2/1 -> Sum5/1
  Transfer Fcn8/1 -> Sum5/2, Scope1/1
  Sum5/1 -> Gain5/1, Transfer Fcn9/1
  Transfer Fcn9/1 -> Sum4/2
  Transfer Fcn7/1 -> Transfer Fcn8/1
  Transfer Fcn15/1 -> Sum8/2
  Constant4/1 -> Sum9/1
  Sum9/1 -> Gain8/1, Transfer Fcn15/1
  Transfer Fcn14/1 -> Gain6/1, Sum9/2, Scope3/1
  Gain8/1 -> Sum8/1
  Transfer Fcn13/1 -> Sum12/2
  Gain10/1 -> Sum12/1
  Sum11/1 -> Gain10/1, Transfer Fcn13/1
  Sum8/1 -> Sum11/1
  Sum12/1 -> Sum10/2
  Sum10/1 -> Transfer Fcn16/1
  Transfer Fcn16/1 -> Sum11/2, Transfer Fcn14/1
  Gain6/1 -> Sum10/1
  Sum15/1 -> Gain9/1, Transfer Fcn11/1
  Gain7/1 -> Sum6/1
  Transfer Fcn10/1 -> Integrator/1, Gain7/1, Sum15/2, Scope2/1
  Transfer Fcn11/1 -> Sum14/2
  Sum6/1 -> Transfer Fcn12/1
  Transfer Fcn12/1 -> Sum7/2, Transfer Fcn10/1
  Gain4/1 -> Sum13/1
  Gain9/1 -> Sum14/1
  Transfer Fcn6/1 -> Sum13/2
  Sum14/1 -> Sum7/1
  Sum7/1 -> Gain4/1, Transfer Fcn6/1
  Sum13/1 -> Sum6/2
  Gain11/1 -> Manual Switch/2, Sum17/2
  Sum16/1 -> Gain11/1
  Sine Wave1/1 -> Gain12/1, Sum16/1
  Integrator/1 -> Scope4/1, Sum16/2
  Gain12/1 -> Derivative2/1
  Derivative2/1 -> Sum17/1
  Manual Switch/1 -> Sum15/1
  Sum17/1 -> Manual Switch/1
  Constant3/1 -> Sum19/1
  Transfer Fcn1/1 -> Transfer Fcn2/1
  PID Controller4/1 -> Transfer Fcn1/1
  Transfer Fcn2/1 -> Sum19/2, Scope5/1
  PID Controller3/1 -> Manual Switch1/2, Sum23/2
  Integrator1/1 -> Scope7/1, Sum22/2
  Transfer Fcn17/1 -> Scope6/1, Sum21/2, Integrator1/1, Gain16/1
  Gain16/1 -> Sum24/1
  PID Controller1/1 -> Sum25/1
  Sum24/1 -> Transfer Fcn19/1
  Transfer Fcn19/1 -> Sum25/2, Transfer Fcn17/1
  Gain14/1 -> Derivative3/1
  Manual Switch1/1 -> Sum21/1
  Sine Wave3/1 -> Gain14/1, Sum22/1
  Derivative3/1 -> Sum23/1
  PID Controller2/1 -> Sum24/2
  Sum25/1 -> PID Controller2/1
  Sum21/1 -> PID Controller1/1
  Sum23/1 -> Manual Switch1/1
  Sum22/1 -> PID Controller3/1
  Sum19/1 -> PID Controller4/1
  Constant6/1 -> Sum20/1
  Transfer Fcn20/1 -> Sum20/2, Scope8/1
  Transfer Fcn18/1 -> Transfer Fcn20/1
  PID Controller5/1 -> Transfer Fcn18/1
  Sum20/1 -> PID Controller5/1
  Sum29/1 -> PID Controller9/1
  Manual Switch2/1 -> Sum18/1
  Sum18/1 -> PID Controller6/1
  PID Controller9/1 -> Sum28/2
  Step9/1 -> Gain13/1, Sum26/1
  PID Controller6/1 -> Sum29/1
  Gain15/1 -> Sum28/1
  Transfer Fcn21/1 -> Scope9/1, Sum18/2, Integrator2/1, Gain15/1
  PID Controller8/1 -> Manual Switch2/2, Sum27/2
  Sum28/1 -> Transfer Fcn22/1
  Transfer Fcn22/1 -> Scope30/1, Sum29/2, Transfer Fcn21/1
  Sum26/1 -> PID Controller8/1
  Sum27/1 -> Manual Switch2/1
  Gain13/1 -> Derivative4/1
  Derivative4/1 -> Sum27/1
  Integrator2/1 -> Scope10/1, Sum26/2
  Rate Transition1/1 -> Speed and Current Loop2/3(ic)
  Constant9/1 -> Mod1/2
  From4/1 -> Data Type Conversion6/1
  Bus Selector2/2 -> Goto6/1  "<IbStator>"
  From7/1 -> Scope15/1
  Data Type Conversion2/1 -> Rate Transition7/1
  Derivative5/1 -> Sum30/2
  Rate Transition2/1 -> Speed and Current Loop2/5(SpeedRef)
  Step1/1 -> Manual Switch7/1
  From8/1 -> Data Type Conversion1/1
  Function-Call Generator1/1 -> PositionLoop1/Trigger
  From1/1 -> Rate Transition5/1
  Sum30/1 -> Manual Switch8/2
  Data Type Conversion1/1 -> Rate Transition6/1
  Gain18/1 -> Goto2/1
  Manual Switch8/1 -> Manual Switch3/2
  Constant11/1 -> Rate Transition3/1
  Rate Transition6/1 -> Speed and Current Loop2/1(ia)
  From9/1 -> Scope24/1
  Rate Transition7/1 -> Speed and Current Loop2/2(ib)
  Constant10/1 -> Average-Value Inverter2/2
  Average-Value Inverter2/1 -> Surface Mount PMSM2/2
  Bus Selector2/1 -> Goto5/1  "<IaStator>"
  From12/1 -> Scope18/1
  Subsystem2/1(DutyOut) -> Average-Value Inverter2/1
  Gain17/1 -> Derivative5/1
  Rate Transition5/1 -> Speed and Current Loop2/7(theta)
  Speed and Current Loop2/1(tABC) -> Subsystem2/1(DutyIn)
  Data Type Conversion6/1 -> Rate Transition1/1
  Bus Selector2/3 -> Goto14/1  "<IcStator>"
  Gain19/1 -> Mod1/1
  rad/s2/1 -> Manual Switch3/1
  From3/1 -> Data Type Conversion2/1
  Sine Wave5/1 -> Manual Switch7/2
  From2/1 -> PositionLoop1/2(PositionFd)
  Surface Mount PMSM2/1 -> Bus Selector2/1
  Rate Transition4/1 -> Speed and Current Loop2/6(SpeedFd)
  Mod1/1 -> Goto1/1
  Rate Transition3/1 -> Speed and Current Loop2/4(v_bus)
  From6/1 -> Scope23/1
  Sum/1 -> PID Controller/1
  State-Space/1 -> Scope25/1, Sum/2
  Step2/1 -> Sum/1
  Step4/1 -> Sum31/1
  State-Space1/1 -> Scope26/1, Sum31/2
  Transfer Fcn23/1 -> Transfer Fcn24/1
  PID Controller10/1 -> Transfer Fcn23/1
  Sum32/1 -> PID Controller10/1
  Transfer Fcn24/1 -> Sum32/2, State-Space1/1
  Step5/1 -> Sum33/1
  Uncertain State Space/1 -> MultiPlot Graph/1, Sum33/2
  State-Space2/1 -> Scope27/1, Sum34/2
  Step6/1 -> Sum34/1
  Sum34/1 -> Transfer Fcn28/1
  Sum33/1 -> Transfer Fcn25/1
  Transfer Fcn25/1 -> Uncertain State Space/1
  Rate Transition14/1 -> Robust control/4(v_bus)
  From14/1 -> Scope31/1
  Data Type Conversion9/1 -> Rate Transition11/1
  From27/1 -> Scope34/1
  Surface Mount PMSM3/1 -> Scope37/1, Bus Selector3/1
  Mod2/1 -> Goto15/1
  Gain22/1 -> Mod2/1
  From24/1 -> Data Type Conversion8/1
  Bus Selector3/3 -> Goto16/1  "<IcStator>"
  From13/1 -> Rate Transition18/1
  Average-Value Inverter3/1 -> Surface Mount PMSM3/2
  Constant13/1 -> Rate Transition14/1
  Bus Selector3/1 -> Goto20/1  "<IaStator>"
  Subsystem3/1(DutyOut) -> Average-Value Inverter3/1
  Rate Transition18/1 -> Robust control/5(theta_e)
  Rate Transition19/1 -> Robust control/1(ia)
  Constant12/1 -> Average-Value Inverter3/2
  From29/1 -> Data Type Conversion7/1
  Data Type Conversion7/1 -> Rate Transition19/1
  Rate Transition20/1 -> Robust control/2(ib)
  Bus Selector3/2 -> Goto21/1  "<IbStator>"
  Robust control/1(tABC) -> Subsystem3/1(DutyIn)
  Data Type Conversion8/1 -> Rate Transition20/1
  Constant14/1 -> Mod2/2
  Bus Selector3/4 -> Goto18/1, Gain40/1, Gain22/1  "<MtrPos>"
  From30/1 -> Scope35/1
  From25/1 -> Data Type Conversion9/1
  Gain21/1 -> Goto17/1
  Surface Mount PMSM3/3 -> Goto19/1, Gain21/1
  Rate Transition11/1 -> Robust control/3(ic)
  Sum31/1 -> Transfer Fcn27/1
  Transfer Fcn27/1 -> Sum32/1
  Manual Switch4/1 -> Scope12/1, Rate Transition13/1
  PositionLoop2/1(SpeedRef) -> Manual Switch6/1, Sum1/1
  Manual Switch5/1 -> Gain/1, PositionLoop2/1(PositionRef), Scope17/1
  From18/1 -> Scope14/1, Rate Transition16/1
  Surface Mount PMSM1/3 -> Goto13/1, Gain2/1
  Bus Selector1/4 -> Goto12/1, Gain3/1  "<MtrPos>"
  Manual Switch3/1 -> Scope16/1, Rate Transition2/1
  PositionLoop1/1(SpeedRef) -> Manual Switch8/1, Sum30/1
  From5/1 -> Scope20/1, Rate Transition4/1
  Manual Switch7/1 -> Scope22/1, PositionLoop1/1(PositionRef), Gain17/1
  Surface Mount PMSM2/3 -> Goto4/1, Gain18/1
  Bus Selector2/4 -> Goto3/1, Gain19/1  "<MtrPos>"
  Sum36/1 -> State-Space/1
  PID Controller/1 -> Sum36/1
  Step10/1 -> Sum36/2
  Transfer Fcn28/1 -> Sum37/1
  Sum37/1 -> State-Space2/1
  Step11/1 -> Sum37/2
  Subsystem5/1(DutyOut) -> Average-Value Inverter5/1
  From45/1 -> Scope28/1
  Bus Selector5/2 -> Goto35/1  "<IbStator>"
  Surface Mount PMSM5/3 -> Goto33/1, Gain25/1
  Data Type Conversion16/1 -> Rate Transition33/1
  Constant18/1 -> Average-Value Inverter5/2
  From39/1 -> Scope40/1
  Sine Wave8/1 -> Manual Switch12/2
  Manual Switch12/1 -> Subsystem6/5(PositionRef), Scope42/1
  Bus Selector5/4 -> Goto32/1, Gain26/1  "<MtrPos>"
  Bus Selector5/1 -> Goto34/1  "<IaStator>"
  Step12/1 -> Manual Switch12/1
  From41/1 -> Data Type Conversion16/1
  Surface Mount PMSM5/1 -> Bus Selector5/1
  Bus Selector5/3 -> Goto30/1  "<IcStator>"
  From44/1 -> Scope43/1
  Gain26/1 -> Mod5/1
  Mod5/1 -> Goto29/1
  Constant19/1 -> Rate Transition29/1
  Data Type Conversion15/1 -> Rate Transition32/1
  From43/1 -> Scope41/1, Rate Transition30/1
  From42/1 -> Data Type Conversion17/1
  Data Type Conversion17/1 -> Rate Transition27/1
  From36/1 -> Rate Transition31/1
  Average-Value Inverter5/1 -> Surface Mount PMSM5/2
  From46/1 -> Data Type Conversion15/1
  Constant20/1 -> Mod5/2
  From47/1 -> Scope44/1
  Gain25/1 -> Goto31/1
  Rate Transition32/1 -> Subsystem6/1(ia)
  Rate Transition33/1 -> Subsystem6/2(ib)
  Rate Transition27/1 -> Subsystem6/3(ic)
  Rate Transition29/1 -> Subsystem6/4(v_bus)
  From40/1 -> Subsystem6/6(PositionFd)
  Rate Transition30/1 -> Subsystem6/7(SpeedFd)
  Rate Transition31/1 -> Subsystem6/8(theta)
  Subsystem6/1(tABC) -> Subsystem5/1(DutyIn)
  Subsystem7/1(DutyOut) -> Average-Value Inverter6/1
  From55/1 -> Scope39/1
  Bus Selector6/2 -> Goto42/1  "<IbStator>"
  Surface Mount PMSM6/3 -> Goto40/1, Gain27/1
  Data Type Conversion19/1 -> Rate Transition39/1
  Constant21/1 -> Average-Value Inverter6/2
  From49/1 -> Scope46/1
  Sine Wave9/1 -> Manual Switch13/2
  Manual Switch13/1 -> Triloop_Feedforward/5(PositionRef), Scope48/1
  Bus Selector6/4 -> Goto39/1, Gain28/1  "<MtrPos>"
  Bus Selector6/1 -> Goto41/1  "<IaStator>"
  Step13/1 -> Manual Switch13/1
  From51/1 -> Data Type Conversion19/1
  Surface Mount PMSM6/1 -> Bus Selector6/1
  Bus Selector6/3 -> Goto37/1  "<IcStator>"
  From54/1 -> Scope49/1
  Gain28/1 -> Mod6/1
  Mod6/1 -> Goto36/1
  Constant22/1 -> Rate Transition35/1
  Data Type Conversion18/1 -> Rate Transition38/1
  From53/1 -> Scope47/1, Rate Transition36/1
  From52/1 -> Data Type Conversion20/1
  Data Type Conversion20/1 -> Rate Transition28/1
  From48/1 -> Rate Transition37/1
  Average-Value Inverter6/1 -> Surface Mount PMSM6/2
  From56/1 -> Data Type Conversion18/1
  Constant23/1 -> Mod6/2
  From57/1 -> Scope50/1
  Gain27/1 -> Goto38/1
  Rate Transition38/1 -> Triloop_Feedforward/1(ia)
  Rate Transition39/1 -> Triloop_Feedforward/2(ib)
  Rate Transition28/1 -> Triloop_Feedforward/3(ic)
  Rate Transition35/1 -> Triloop_Feedforward/4(v_bus)
  From50/1 -> Triloop_Feedforward/6(PositionFd)
  Rate Transition36/1 -> Triloop_Feedforward/7(SpeedFd)
  Rate Transition37/1 -> Triloop_Feedforward/8(theta)
  Triloop_Feedforward/1(tABC) -> Subsystem7/1(DutyIn)
  Gain31/1 -> Derivative14/1
  Derivative14/1 -> Derivative15/1
  Derivative17/1 -> Derivative11/1
  Gain33/1 -> Derivative13/1
  Derivative15/1 -> Derivative16/1
  Gain32/1 -> Derivative17/1
  Sum40/1 -> Gain38/1, Transfer Fcn32/1
  Manual Switch11/1 -> Sum40/1
  Sum43/1 -> Transfer Fcn33/1
  Sum39/1 -> Sum44/1
  Add/1 -> Sum42/1
  Sum38/1 -> Sum43/2
  Sine Wave10/1 -> Sum41/1, Gain30/1, Gain35/1, Gain34/1
  Gain24/1 -> Manual Switch11/2, Sum42/2
  Transfer Fcn33/1 -> Sum44/2, Transfer Fcn31/1
  Gain38/1 -> Sum39/1
  Sum41/1 -> Gain24/1
  Transfer Fcn34/1 -> Sum38/2
  Sum42/1 -> Manual Switch11/1
  Transfer Fcn32/1 -> Sum39/2
  Transfer Fcn31/1 -> Integrator3/1, Gain37/1, Sum40/2, Scope45/1
  Gain36/1 -> Sum38/1
  Sum44/1 -> Gain36/1, Transfer Fcn34/1
  Gain34/1 -> Derivative12/1
  Integrator3/1 -> Scope51/1, Sum41/2
  Gain37/1 -> Sum43/1
  Derivative9/1 -> Derivative10/1
  Derivative8/1 -> Derivative9/1
  Gain35/1 -> Derivative7/1
  Gain30/1 -> Derivative8/1
  Derivative12/1 -> Derivative6/1
  Derivative10/1 -> Add/3
  Derivative6/1 -> Add/2
  Derivative7/1 -> Add/1
  Derivative18/1 -> Sum47/1
  Gain39/1 -> Sum48/1
  Integrator4/1 -> Scope52/1, Sum46/2
  PID Controller13/1 -> Manual Switch14/2, Sum47/2
  Step14/1 -> Gain29/1, Sum46/1
  Gain29/1 -> Derivative18/1
  Transfer Fcn36/1 -> Scope53/1, Sum49/2, Transfer Fcn35/1
  Sum48/1 -> Transfer Fcn36/1
  Sum46/1 -> PID Controller13/1
  Manual Switch14/1 -> Sum49/1
  Sum49/1 -> PID Controller12/1
  Transfer Fcn35/1 -> Scope54/1, Integrator4/1, Gain39/1
  Sum47/1 -> Manual Switch14/1
  PID Controller12/1 -> Sum48/2
  Gain40/1 -> Mod7/1
  Constant24/1 -> Mod7/2
  Mod7/1 -> Goto43/1
  From58/1 -> Scope55/1
  Step8/1 -> Sum50/2
  Step15/1 -> Sum45/1
  State-Space3/1 -> Scope29/1, Sum45/2
  Sum45/1 -> Transfer Fcn26/1
  Transfer Fcn26/1 -> Scope32/1, Sum50/1
  Sum50/1 -> State-Space3/1
  Subsystem4/1(DutyOut) -> Average-Value Inverter4/1
  From33/1 -> Data Type Conversion14/1
  Surface Mount PMSM4/3 -> Goto26/1, Gain20/1
  Constant16/1 -> Rate Transition23/1
  Average-Value Inverter4/1 -> Surface Mount PMSM4/2
  Rate Transition25/1 -> Speed and Current Loop4/1(ia)
  Bus Selector4/3 -> Goto23/1  "<IcStator>"
  Data Type Conversion13/1 -> Rate Transition26/1
  Gain20/1 -> Goto24/1
  Rate Transition26/1 -> Speed and Current Loop4/2(ib)
  From32/1 -> Data Type Conversion13/1
  From26/1 -> Rate Transition24/1
  Data Type Conversion14/1 -> Rate Transition17/1
  Step16/1 -> Speed and Current Loop4/6(theta_ref)
  Mod4/1 -> Goto22/1
  Speed and Current Loop4/1(tABC) -> Subsystem4/1(DutyIn)
  From35/1 -> Data Type Conversion12/1
  Constant15/1 -> Average-Value Inverter4/2
  Bus Selector4/1 -> Goto27/1  "<IaStator>"
  Data Type Conversion12/1 -> Rate Transition25/1
  Constant17/1 -> Mod4/2
  Rate Transition23/1 -> Speed and Current Loop4/4(v_bus)
  Bus Selector4/4 -> Goto/1, Gain23/1  "<MtrPos>"
  Gain23/1 -> Mod4/1
  From37/1 -> Scope56/1
  Surface Mount PMSM4/1 -> Bus Selector4/1
  Rate Transition17/1 -> Speed and Current Loop4/3(ic)
  Bus Selector4/2 -> Goto28/1  "<IbStator>"
  Rate Transition24/1 -> Speed and Current Loop4/5(theta)
  From28/1 -> Scope36/1
  From34/1 -> Scope38/1
  From31/1 -> Speed and Current Loop4/7(theta_m)
  From15/1 -> Robust control/9(theta_output)
  Step7/1 -> Robust control/8(theta_ref)
  Constant25/1 -> Robust control/6(P)
  Constant26/1 -> Robust control/7(I)
  Transfer Fcn37/1 -> Sum51/1
  Sum35/1 -> Transfer Fcn37/1
  Sum51/1 -> PID Controller7/1
  State-Space4/1 -> Scope33/1, Sum35/2
  PID Controller7/1 -> Transfer Fcn29/1
  Transfer Fcn30/1 -> Sum51/2, State-Space4/1
  Transfer Fcn29/1 -> Transfer Fcn30/1
  Step17/1 -> Sum35/1
  Sum52/1 -> Transfer Fcn40/1
  Step18/1 -> Sum52/1
  State-Space5/1 -> Scope57/1, Sum52/2
  Transfer Fcn39/1 -> State-Space5/1
  Transfer Fcn40/1 -> Transfer Fcn39/1
